simulink model "CIC2026_C1"  (R2025b)
settings: Solver=ode45  StartTime=0.0  StopTime=8000  FixedStep=0.1  RelTol=1e-3
StopFcn:
  | GuardaResultadoSimulacion;
model workspace (MATLAB code in the model file):
  | % 24 ºC
  | %%%%%%%%%%%%%%%%%%%%%%%%%%%%%%%%%%%%%%%%%%%%%%%%%%
  | Tev_Qev_24_75 = ...
  | [5.0,37.938;
  | 5.1,37.939 ;
  | 5.2,38.028 ;
  | 5.3,38.162 ;
  | 5.4,38.43  ;
  | 5.5,38.698 ;
  | 5.6,38.839 ;
  | 5.7,38.89  ;
  | 5.8,38.941 ;
  | 5.9,38.992 ;
  | 6,39.043   ;
  | 6.1,38.997 ;
  | 6.2,38.942 ;
  | 6.3,38.887 ;
  | 6.4,38.832 ;
  | 6.5,39.018 ;
  | 6.6,39.375 ;
  | 6.7,39.65  ;
  | 6.8,39.679 ;
  | 6.9,39.707 ;
  | 7,39.736   ;
  | 7.1,39.745 ;
  | 7.2,39.643 ;
  | 7.3,39.643 ;
  | 7.4,39.643 ;
  | 7.5,39.643 ;
  | 7.6,39.643 ;
  | 7.7,39.643 ;
  | 7.8,39.643 ;
  | 7.9,39.643 ;
  | 8,39.643   ;
  | 8.1,39.643 ;
  | 8.2,39.643 ;
  | 8.3,39.643 ;
  | 8.4,39.643 ;
  | 8.5,39.643 ;
  | 8.6,39.643 ;
  | 8.7,39.643 ;
  | 8.8,39.643 ;
  | 8.9,39.643 ;
  | 9,39.643   ;
  | 9.1,39.643 ;
  | 9.2,39.643 ;
  | 9.3,39.643 ;
  | 9.4,39.643 ;
  | 9.5,39.643 ;
  | 9.6,39.643 ;
  | 9.7,39.643 ;
  | 9.8,39.643 ;
  | 9.9,39.643 ;
  | 10,39.642  ;
  | 10.1,39.636;
  | 10.2,39.63 ;
  | 10.3,39.624;
  | 10.4,39.618;
  | 10.5,39.612;
  | 10.6,39.606;
  | 10.7,39.601;
  | 10.8,39.595;
  | 10.9,39.589;
  | 11,39.583  ;
  | 11.1,39.577;
  | 11.2,39.571;
  | 11.3,39.565;
  | 11.4,39.559;
  | 11.5,39.553;
  | 11.6,39.547;
  | 11.7,39.541;
  | 11.8,39.535;
  | 11.9,39.529;
  | 12.0,39.529];
  | 
  | Tev_Qev_24_80 = ...
  | [
  | 5.0,40.849   ;
  | 5.1,41.042   ;
  | 5.2,41.236   ;
  | 5.3,41.429   ;
  | 5.4,41.786   ;
  | 5.5,42.143   ;
  | 5.6,42.391   ;
  | 5.7,42.585   ;
  | 5.8,42.778   ;
  | 5.9,42.972   ;
  | 6,43.166     ;
  | 6.1,43.363   ;
  | 6.2,43.562   ;
  | 6.3,43.761   ;
  | 6.4,43.96    ;
  | 6.5,44.158   ;
  | 6.6,44.357   ;
  | 6.7,44.556   ;
  | 6.8,44.755   ;
  | 6.9,44.953   ;
  | 7,45.159     ;
  | 7.1,45.397   ;
  | 7.2,45.6     ;
  | 7.3,45.628   ;
  | 7.4,45.656   ;
  | 7.5,45.684   ;
  | 7.6,45.712   ;
  | 7.7,45.119   ;
  | 7.8,45.119   ;
  | 7.9,45.119   ;
  | 8,45.119     ;
  | 8.1,45.109   ;
  | 8.2,45.097   ;
  | 8.3,45.085   ;
  | 8.4,45.073   ;
  | 8.5,45.061   ;
  | 8.6,45.049   ;
  | 8.7,45.037   ;
  | 8.8,45.025   ;
  | 8.9,45.013   ;
  | 9,45.001     ;
  | 9.1,45.011   ;
  | 9.2,45.023   ;
  | 9.3,45.035   ;
  | 9.4,45.047   ;
  | 9.5,45.059   ;
  | 9.6,45.07    ;
  | 9.7,45.082   ;
  | 9.8,45.094   ;
  | 9.9,45.106   ;
  | 10,45.118    ;
  | 10.1,45.108  ;
  | 10.2,45.096  ;
  | 10.3,45.084  ;
  | 10.4,45.072  ;
  | 10.5,45.06   ;
  | 10.6,45.048  ;
  | 10.7,45.036  ;
  | 10.8,45.024  ;
  | 10.9,45.012  ;
  | 11,45        ;
  | 11.1,45.012  ;
  | 11.2,45.024  ;
  | 11.3,45.036  ;
  | 11.4,45.048  ;
  | 11.5,45.061  ;
  | 11.6,45.073  ;
  | 11.7,45.085  ;
  | 11.8,45.097  ;
  | 11.9,45.109  ;
  | 12.0,45.109
  | ];
  | 
  | Tev_Qev_24_85 = ...
  | [
  | 5.0,41.595   ;
  | 5.1,42.167   ;
  | 5.2,42.659   ;
  | 5.3,43.135   ;
  | 5.4,43.611   ;
  | 5.5,44.087   ;
  | 5.6,44.544   ;
  | 5.7,44.996   ;
  | 5.8,45.448   ;
  | 5.9,45.901   ;
  | 6,46.353     ;
  | 6.1,46.776   ;
  | 6.2,47.192   ;
  | 6.3,47.609   ;
  | 6.4,48.026   ;
  | 6.5,48.442   ;
  | 6.6,48.859   ;
  | 6.7,49.276   ;
  | 6.8,49.692   ;
  | 6.9,50       ;
  | 7,50.299     ;
  | 7.1,50.667   ;
  | 7.2,51.034   ;
  | 7.3,51.345   ;
  | 7.4,51.534   ;
  | 7.5,51.786   ;
  | 7.6,51.786   ;
  | 7.7,51.786   ;
  | 7.8,51.786   ;
  | 7.9,51.786   ;
  | 8,51.786     ;
  | 8.1,51.776   ;
  | 8.2,51.764   ;
  | 8.3,51.752   ;
  | 8.4,51.74    ;
  | 8.5,51.728   ;
  | 8.6,51.716   ;
  | 8.7,51.704   ;
  | 8.8,51.692   ;
  | 8.9,51.68    ;
  | 9,51.668     ;
  | 9.1,51.688   ;
  | 9.2,51.711   ;
  | 9.3,51.734   ;
  | 9.4,51.757   ;
  | 9.5,51.78    ;
  | 9.6,51.905   ;
  | 9.7,52.063   ;
  | 9.8,52.222   ;
  | 9.9,52.254   ;
  | 10,52.244    ;
  | 10.1,52.234  ;
  | 10.2,52.223  ;
  | 10.3,52.213  ;
  | 10.4,52.203  ;
  | 10.5,52.193  ;
  | 10.6,52.182  ;
  | 10.7,52.172  ;
  | 10.8,52.162  ;
  | 10.9,52.151  ;
  | 11,52.147    ;
  | 11.1,52.171  ;
  | 11.2,52.195  ;
  | 11.3,52.219  ;
  | 11.4,52.243  ;
  | 11.5,52.267  ;
  | 11.6,52.291  ;
  | 11.7,52.315  ;
  | 11.8,52.339  ;
  | 11.9,52.363  ;
  | 12.0,52.363
  | ];
  | 
  | Tev_Qev_24_88 = ...
  | [
  | 5,44.09      ;
  | 5.1,44.594   ;
  | 5.2,44.992   ;
  | 5.3,45.337   ;
  | 5.4,45.774   ;
  | 5.5,46.488   ;
  | 5.6,47.168   ;
  | 5.7,47.47    ;
  | 5.8,47.772   ;
  | 5.9,48.075   ;
  | 6,48.377     ;
  | 6.1,48.759   ;
  | 6.2,49.167   ;
  | 6.3,49.325   ;
  | 6.4,49.484   ;
  | 6.5,49.952   ;
  | 6.6,50.524   ;
  | 6.7,50.994   ;
  | 6.8,51.162   ;
  | 6.9,51.331   ;
  | 7,51.634     ;
  | 7.1,52.126   ;
  | 7.2,52.619   ;
  | 7.3,53.016   ;
  | 7.4,53.506   ;
  | 7.5,54.091   ;
  | 7.6,54.286   ;
  | 7.7,54.568   ;
  | 7.8,54.991   ;
  | 7.9,55.238   ;
  | 8,55.238     ;
  | 8.1,55.238   ;
  | 8.2,55.506   ;
  | 8.3,55.595   ;
  | 8.4,55.595   ;
  | 8.5,55.595   ;
  | 8.6,55.595   ;
  | 8.7,55.595   ;
  | 8.8,55.595   ;
  | 8.9,55.595   ;
  | 9,55.595     ;
  | 9.1,55.595   ;
  | 9.2,55.595   ;
  | 9.3,55.595   ;
  | 9.4,55.595   ;
  | 9.5,55.608   ;
  | 9.6,55.767   ;
  | 9.7,55.926   ;
  | 9.8,56.071   ;
  | 9.9,56.071   ;
  | 10,56.071    ;
  | 10.1,56.071  ;
  | 10.2,56.071  ;
  | 10.3,56.071  ;
  | 10.4,56.071  ;
  | 10.5,56.071  ;
  | 10.6,56.071  ;
  | 10.7,56.071  ;
  | 10.8,56.071  ;
  | 10.9,56.071  ;
  | 11,56.071    ;
  | 11.1,56.071  ;
  | 11.2,56.071  ;
  | 11.3,56.071  ;
  | 11.4,56.071  ;
  | 11.5,56.071  ;
  | 11.6,56.071  ;
  | 11.7,56.071  ;
  | 11.8,56.071  ;
  | 11.9,56.071  ;
  | 12.0,56.071
  | ];
  | 
  | Tev_Qev_24_95 = ...
  | [
  | 5,46.228     ;
  | 5.1,46.674   ;
  | 5.2,47.121   ;
  | 5.3,47.567   ;
  | 5.4,48.019   ;
  | 5.5,48.529   ;
  | 5.6,49.039   ;
  | 5.7,49.549   ;
  | 5.8,50.081   ;
  | 5.9,50.627   ;
  | 6,51.173     ;
  | 6.1,51.778   ;
  | 6.2,52.403   ;
  | 6.3,53.028   ;
  | 6.4,53.653   ;
  | 6.5,54.039   ;
  | 6.6,54.345   ;
  | 6.7,54.821   ;
  | 6.8,55.536   ;
  | 6.9,56.221   ;
  | 7,56.584     ;
  | 7.1,56.948   ;
  | 7.2,57.312   ;
  | 7.3,57.675   ;
  | 7.4,58       ;
  | 7.5,58.286   ;
  | 7.6,58.552   ;
  | 7.7,58.746   ;
  | 7.8,58.832   ;
  | 7.9,58.865   ;
  | 8,58.898     ;
  | 8.1,58.96    ;
  | 8.2,59.332   ;
  | 8.3,59.637   ;
  | 8.4,59.599   ;
  | 8.5,59.561   ;
  | 8.6,59.524   ;
  | 8.7,59.646   ;
  | 8.8,59.768   ;
  | 8.9,59.89    ;
  | 9,60.012     ;
  | 9.1,60.134   ;
  | 9.2,60.256   ;
  | 9.3,60.363   ;
  | 9.4,60.395   ;
  | 9.5,60.427   ;
  | 9.6,60.46    ;
  | 9.7,60.563   ;
  | 9.8,60.738   ;
  | 9.9,60.912   ;
  | 10,61.068    ;
  | 10.1,61.028  ;
  | 10.2,60.989  ;
  | 10.3,60.949  ;
  | 10.4,60.909  ;
  | 10.5,60.87   ;
  | 10.6,60.833  ;
  | 10.7,60.833  ;
  | 10.8,60.833  ;
  | 10.9,60.833  ;
  | 11,60.832    ;
  | 11.1,60.82   ;
  | 11.2,60.808  ;
  | 11.3,60.796  ;
  | 11.4,60.784  ;
  | 11.5,60.772  ;
  | 11.6,60.76   ;
  | 11.7,60.748  ;
  | 11.8,60.735  ;
  | 11.9,60.723  ;
  | 12.0,60.723
  | ];
  | 
  | Tev_COP_24_75 = ...
  | [
  | 5,0.704      ;
  | 5.1,0.708    ;
  | 5.2,0.712    ;
  | 5.3,0.716    ;
  | 5.4,0.72     ;
  | 5.5,0.724    ;
  | 5.6,0.728    ;
  | 5.7,0.732    ;
  | 5.8,0.736    ;
  | 5.9,0.74     ;
  | 6,0.743      ;
  | 6.1,0.747    ;
  | 6.2,0.752    ;
  | 6.3,0.758    ;
  | 6.4,0.765    ;
  | 6.5,0.77     ;
  | 6.6,0.774    ;
  | 6.7,0.777    ;
  | 6.8,0.779    ;
  | 6.9,0.781    ;
  | 7,0.788      ;
  | 7.1,0.794    ;
  | 7.2,0.796    ;
  | 7.3,0.796    ;
  | 7.4,0.796    ;
  | 7.5,0.796    ;
  | 7.6,0.796    ;
  | 7.7,0.796    ;
  | 7.8,0.796    ;
  | 7.9,0.796    ;
  | 8,0.796      ;
  | 8.1,0.796    ;
  | 8.2,0.796    ;
  | 8.3,0.796    ;
  | 8.4,0.796    ;
  | 8.5,0.797    ;
  | 8.6,0.797    ;
  | 8.7,0.797    ;
  | 8.8,0.797    ;
  | 8.9,0.797    ;
  | 9,0.797      ;
  | 9.1,0.797    ;
  | 9.2,0.797    ;
  | 9.3,0.797    ;
  | 9.4,0.797    ;
  | 9.5,0.797    ;
  | 9.6,0.797    ;
  | 9.7,0.797    ;
  | 9.8,0.797    ;
  | 9.9,0.797    ;
  | 10,0.797     ;
  | 10.1,0.797   ;
  | 10.2,0.798   ;
  | 10.3,0.798   ;
  | 10.4,0.798   ;
  | 10.5,0.798   ;
  | 10.6,0.798   ;
  | 10.7,0.798   ;
  | 10.8,0.798   ;
  | 10.9,0.798   ;
  | 11,0.798     ;
  | 11.1,0.798   ;
  | 11.2,0.798   ;
  | 11.3,0.798   ;
  | 11.4,0.798   ;
  | 11.5,0.798   ;
  | 11.6,0.798   ;
  | 11.7,0.798   ;
  | 11.8,0.798   ;
  | 11.9,0.799   ;
  | 12.0,0.799
  | ];
  | 
  | Tev_COP_24_80 = ...
  | [
  | 5,0.671      ;
  | 5.1,0.677    ;
  | 5.2,0.682    ;
  | 5.3,0.688    ;
  | 5.4,0.693    ;
  | 5.5,0.699    ;
  | 5.6,0.704    ;
  | 5.7,0.709    ;
  | 5.8,0.714    ;
  | 5.9,0.719    ;
  | 6,0.724      ;
  | 6.1,0.728    ;
  | 6.2,0.733    ;
  | 6.3,0.739    ;
  | 6.4,0.743    ;
  | 6.5,0.748    ;
  | 6.6,0.752    ;
  | 6.7,0.758    ;
  | 6.8,0.763    ;
  | 6.9,0.767    ;
  | 7,0.77       ;
  | 7.1,0.773    ;
  | 7.2,0.774    ;
  | 7.3,0.775    ;
  | 7.4,0.775    ;
  | 7.5,0.775    ;
  | 7.6,0.775    ;
  | 7.7,0.776    ;
  | 7.8,0.769    ;
  | 7.9,0.769    ;
  | 8,0.77       ;
  | 8.1,0.77     ;
  | 8.2,0.77     ;
  | 8.3,0.77     ;
  | 8.4,0.769    ;
  | 8.5,0.769    ;
  | 8.6,0.769    ;
  | 8.7,0.769    ;
  | 8.8,0.769    ;
  | 8.9,0.769    ;
  | 9,0.769      ;
  | 9.1,0.769    ;
  | 9.2,0.769    ;
  | 9.3,0.769    ;
  | 9.4,0.769    ;
  | 9.5,0.769    ;
  | 9.6,0.769    ;
  | 9.7,0.77     ;
  | 9.8,0.77     ;
  | 9.9,0.77     ;
  | 10,0.77      ;
  | 10.1,0.77    ;
  | 10.2,0.77    ;
  | 10.3,0.77    ;
  | 10.4,0.77    ;
  | 10.5,0.77    ;
  | 10.6,0.77    ;
  | 10.7,0.77    ;
  | 10.8,0.77    ;
  | 10.9,0.77    ;
  | 11,0.77      ;
  | 11.1,0.77    ;
  | 11.2,0.77    ;
  | 11.3,0.77    ;
  | 11.4,0.771   ;
  | 11.5,0.771   ;
  | 11.6,0.771   ;
  | 11.7,0.771   ;
  | 11.8,0.771   ;
  | 11.9,0.771   ;
  | 12.0,0.771
  | ];
  | 
  | Tev_COP_24_85 = ...
  | [
  | 5,0.616      ;
  | 5.1,0.622    ;
  | 5.2,0.629    ;
  | 5.3,0.635    ;
  | 5.4,0.641    ;
  | 5.5,0.648    ;
  | 5.6,0.654    ;
  | 5.7,0.66     ;
  | 5.8,0.666    ;
  | 5.9,0.671    ;
  | 6,0.675      ;
  | 6.1,0.68     ;
  | 6.2,0.686    ;
  | 6.3,0.691    ;
  | 6.4,0.697    ;
  | 6.5,0.702    ;
  | 6.6,0.708    ;
  | 6.7,0.713    ;
  | 6.8,0.719    ;
  | 6.9,0.724    ;
  | 7,0.73       ;
  | 7.1,0.734    ;
  | 7.2,0.738    ;
  | 7.3,0.741    ;
  | 7.4,0.742    ;
  | 7.5,0.742    ;
  | 7.6,0.742    ;
  | 7.7,0.742    ;
  | 7.8,0.742    ;
  | 7.9,0.743    ;
  | 8,0.743      ;
  | 8.1,0.743    ;
  | 8.2,0.743    ;
  | 8.3,0.742    ;
  | 8.4,0.742    ;
  | 8.5,0.742    ;
  | 8.6,0.742    ;
  | 8.7,0.742    ;
  | 8.8,0.742    ;
  | 8.9,0.742    ;
  | 9,0.743      ;
  | 9.1,0.745    ;
  | 9.2,0.746    ;
  | 9.3,0.746    ;
  | 9.4,0.747    ;
  | 9.5,0.747    ;
  | 9.6,0.747    ;
  | 9.7,0.748    ;
  | 9.8,0.748    ;
  | 9.9,0.748    ;
  | 10,0.749     ;
  | 10.1,0.748   ;
  | 10.2,0.748   ;
  | 10.3,0.748   ;
  | 10.4,0.748   ;
  | 10.5,0.748   ;
  | 10.6,0.748   ;
  | 10.7,0.748   ;
  | 10.8,0.747   ;
  | 10.9,0.747   ;
  | 11,0.747     ;
  | 11.1,0.747   ;
  | 11.2,0.747   ;
  | 11.3,0.748   ;
  | 11.4,0.748   ;
  | 11.5,0.748   ;
  | 11.6,0.748   ;
  | 11.7,0.748   ;
  | 11.8,0.748   ;
  | 11.9,0.748   ;
  | 12.0,0.748
  | ];
  | 
  | Tev_COP_24_88 = ...
  | [
  | 5,0.601      ;
  | 5.1,0.605    ;
  | 5.2,0.609    ;
  | 5.3,0.613    ;
  | 5.4,0.617    ;
  | 5.5,0.62     ;
  | 5.6,0.624    ;
  | 5.7,0.629    ;
  | 5.8,0.635    ;
  | 5.9,0.64     ;
  | 6,0.646      ;
  | 6.1,0.651    ;
  | 6.2,0.656    ;
  | 6.3,0.66     ;
  | 6.4,0.665    ;
  | 6.5,0.671    ;
  | 6.6,0.678    ;
  | 6.7,0.685    ;
  | 6.8,0.69     ;
  | 6.9,0.695    ;
  | 7,0.7        ;
  | 7.1,0.701    ;
  | 7.2,0.701    ;
  | 7.3,0.704    ;
  | 7.4,0.709    ;
  | 7.5,0.705    ;
  | 7.6,0.703    ;
  | 7.7,0.703    ;
  | 7.8,0.702    ;
  | 7.9,0.702    ;
  | 8,0.702      ;
  | 8.1,0.702    ;
  | 8.2,0.701    ;
  | 8.3,0.701    ;
  | 8.4,0.701    ;
  | 8.5,0.701    ;
  | 8.6,0.701    ;
  | 8.7,0.7      ;
  | 8.8,0.7      ;
  | 8.9,0.702    ;
  | 9,0.705      ;
  | 9.1,0.708    ;
  | 9.2,0.708    ;
  | 9.3,0.708    ;
  | 9.4,0.708    ;
  | 9.5,0.708    ;
  | 9.6,0.708    ;
  | 9.7,0.708    ;
  | 9.8,0.707    ;
  | 9.9,0.707    ;
  | 10,0.707     ;
  | 10.1,0.707   ;
  | 10.2,0.707   ;
  | 10.3,0.707   ;
  | 10.4,0.707   ;
  | 10.5,0.707   ;
  | 10.6,0.707   ;
  | 10.7,0.707   ;
  | 10.8,0.707   ;
  | 10.9,0.707   ;
  | 11,0.707     ;
  | 11.1,0.707   ;
  | 11.2,0.707   ;
  | 11.3,0.708   ;
  | 11.4,0.708   ;
  | 11.5,0.708   ;
  | 11.6,0.708   ;
  | 11.7,0.708   ;
  | 11.8,0.708   ;
  | 11.9,0.708   ;
  | 12.0,0.708
  | ];
  | 
  | Tev_COP_24_95 = ...
  | [
  | 5,0.54        ;
  | 5.1,0.547     ;
  | 5.2,0.555     ;
  | 5.3,0.562     ;
  | 5.4,0.563     ;
  | 5.5,0.565     ;
  | 5.6,0.57      ;
  | 5.7,0.577     ;
  | 5.8,0.584     ;
  | 5.9,0.591     ;
  | 6,0.598       ;
  | 6.1,0.605     ;
  | 6.2,0.609     ;
  | 6.3,0.613     ;
  | 6.4,0.617     ;
  | 6.5,0.621     ;
  | 6.6,0.624     ;
  | 6.7,0.629     ;
  | 6.8,0.638     ;
  | 6.9,0.646     ;
  | 7,0.651       ;
  | 7.1,0.657     ;
  | 7.2,0.662     ;
  | 7.3,0.663     ;
  | 7.4,0.667     ;
  | 7.5,0.672     ;
  | 7.6,0.679     ;
  | 7.7,0.68      ;
  | 7.8,0.68      ;
  | 7.9,0.681     ;
  | 8,0.685       ;
  | 8.1,0.686     ;
  | 8.2,0.686     ;
  | 8.3,0.686     ;
  | 8.4,0.687     ;
  | 8.5,0.687     ;
  | 8.6,0.687     ;
  | 8.7,0.689     ;
  | 8.8,0.691     ;
  | 8.9,0.693     ;
  | 9,0.692       ;
  | 9.1,0.692     ;
  | 9.2,0.691     ;
  | 9.3,0.691     ;
  | 9.4,0.69      ;
  | 9.5,0.689     ;
  | 9.6,0.689     ;
  | 9.7,0.69      ;
  | 9.8,0.692     ;
  | 9.9,0.694     ;
  | 10,0.696      ;
  | 10.1,0.696    ;
  | 10.2,0.695    ;
  | 10.3,0.695    ;
  | 10.4,0.695    ;
  | 10.5,0.695    ;
  | 10.6,0.695    ;
  | 10.7,0.695    ;
  | 10.8,0.695    ;
  | 10.9,0.694    ;
  | 11,0.694      ;
  | 11.1,0.694    ;
  | 11.2,0.694    ;
  | 11.3,0.694    ;
  | 11.4,0.694    ;
  | 11.5,0.694    ;
  | 11.6,0.694    ;
  | 11.7,0.694    ;
  | 11.8,0.694    ;
  | 11.9,0.694    ;
  | 12.0,0.694
  | ];
  | 
  | 
  | % 29 ºC
  | %%%%%%%%%%%%%%%%%%%%%%%%%%%%%%%%%%%%%%%%%%%%%%%%%%
  | Tev_Qev_29_75 = ...
  | [
  | 5,20.985      ;
  | 5.1,21.03     ;
  | 5.2,21.05     ;
  | 5.3,21.069    ;
  | 5.4,21.089    ;
  | 5.5,21.109    ;
  | 5.6,21.128    ;
  | 5.7,21.186    ;
  | 5.8,21.247    ;
  | 5.9,21.308    ;
  | 6,21.366      ;
  | 6.1,21.366    ;
  | 6.2,21.366    ;
  | 6.3,21.366    ;
  | 6.4,21.366    ;
  | 6.5,21.366    ;
  | 6.6,21.366    ;
  | 6.7,21.425    ;
  | 6.8,21.734    ;
  | 6.9,22.044    ;
  | 7,22.074      ;
  | 7.1,22.074    ;
  | 7.2,22.063    ;
  | 7.3,22.049    ;
  | 7.4,22.036    ;
  | 7.5,22.023    ;
  | 7.6,22.009    ;
  | 7.7,21.996    ;
  | 7.8,21.983    ;
  | 7.9,21.969    ;
  | 8,21.956      ;
  | 8.1,21.92     ;
  | 8.2,21.885    ;
  | 8.3,21.85     ;
  | 8.4,21.814    ;
  | 8.5,21.779    ;
  | 8.6,21.744    ;
  | 8.7,21.708    ;
  | 8.8,21.673    ;
  | 8.9,21.638    ;
  | 9,21.602      ;
  | 9.1,21.626    ;
  | 9.2,21.65     ;
  | 9.3,21.674    ;
  | 9.4,21.698    ;
  | 9.5,21.722    ;
  | 9.6,21.747    ;
  | 9.7,21.771    ;
  | 9.8,21.795    ;
  | 9.9,21.819    ;
  | 10,21.84      ;
  | 10.1,21.852   ;
  | 10.2,21.864   ;
  | 10.3,21.876   ;
  | 10.4,21.887   ;
  | 10.5,21.899   ;
  | 10.6,21.911   ;
  | 10.7,21.922   ;
  | 10.8,21.934   ;
  | 10.9,21.946   ;
  | 11,21.956     ;
  | 11.1,21.956   ;
  | 11.2,21.956   ;
  | 11.3,21.956   ;
  | 11.4,21.956   ;
  | 11.5,21.956   ;
  | 11.6,21.956   ;
  | 11.7,21.956   ;
  | 11.8,21.956   ;
  | 11.9,21.956   ;
  | 12,21.946
  | ];
  | 
  | Tev_Qev_29_80 = ...
  | [
  | 5,26.088      ;
  | 5.1,26.243    ;
  | 5.2,26.399    ;
  | 5.3,26.554    ;
  | 5.4,26.71     ;
  | 5.5,26.865    ;
  | 5.6,27.021    ;
  | 5.7,27.177    ;
  | 5.8,27.332    ;
  | 5.9,27.488    ;
  | 6,27.652      ;
  | 6.1,27.872    ;
  | 6.2,28.093    ;
  | 6.3,28.313    ;
  | 6.4,28.533    ;
  | 6.5,28.754    ;
  | 6.6,28.974    ;
  | 6.7,29.194    ;
  | 6.8,29.415    ;
  | 6.9,29.635    ;
  | 7,29.855      ;
  | 7.1,29.865    ;
  | 7.2,29.865    ;
  | 7.3,29.865    ;
  | 7.4,29.865    ;
  | 7.5,29.865    ;
  | 7.6,29.865    ;
  | 7.7,29.865    ;
  | 7.8,29.865    ;
  | 7.9,29.865    ;
  | 8,29.865      ;
  | 8.1,29.865    ;
  | 8.2,29.865    ;
  | 8.3,29.865    ;
  | 8.4,29.865    ;
  | 8.5,29.865    ;
  | 8.6,29.865    ;
  | 8.7,29.865    ;
  | 8.8,29.865    ;
  | 8.9,29.865    ;
  | 9,29.865      ;
  | 9.1,29.865    ;
  | 9.2,29.865    ;
  | 9.3,29.865    ;
  | 9.4,29.865    ;
  | 9.5,29.865    ;
  | 9.6,29.865    ;
  | 9.7,29.865    ;
  | 9.8,29.865    ;
  | 9.9,29.865    ;
  | 10,29.864     ;
  | 10.1,29.852   ;
  | 10.2,29.84    ;
  | 10.3,29.828   ;
  | 10.4,29.817   ;
  | 10.5,29.805   ;
  | 10.6,29.793   ;
  | 10.7,29.781   ;
  | 10.8,29.769   ;
  | 10.9,29.758   ;
  | 11,29.746     ;
  | 11.1,29.734   ;
  | 11.2,29.722   ;
  | 11.3,29.711   ;
  | 11.4,29.699   ;
  | 11.5,29.687   ;
  | 11.6,29.675   ;
  | 11.7,29.663   ;
  | 11.8,29.652   ;
  | 11.9,29.64    ;
  | 12,29.629
  | ];
  | 
  | Tev_Qev_29_85 = ...
  | [
  | 5,27.071      ;
  | 5.1,27.57     ;
  | 5.2,28.043    ;
  | 5.3,28.504    ;
  | 5.4,29.053    ;
  | 5.5,29.661    ;
  | 5.6,30.258    ;
  | 5.7,30.737    ;
  | 5.8,31.215    ;
  | 5.9,31.694    ;
  | 6,32.161      ;
  | 6.1,32.551    ;
  | 6.2,32.941    ;
  | 6.3,33.331    ;
  | 6.4,33.722    ;
  | 6.5,34.112    ;
  | 6.6,34.577    ;
  | 6.7,34.972    ;
  | 6.8,35.331    ;
  | 6.9,35.707    ;
  | 7,36.089      ;
  | 7.1,36.471    ;
  | 7.2,36.817    ;
  | 7.3,36.603    ;
  | 7.4,37.299    ;
  | 7.5,37.279    ;
  | 7.6,37.26     ;
  | 7.7,37.241    ;
  | 7.8,37.222    ;
  | 7.9,37.203    ;
  | 8,37.184      ;
  | 8.1,37.17     ;
  | 8.2,37.157    ;
  | 8.3,37.144    ;
  | 8.4,37.13     ;
  | 8.5,37.117    ;
  | 8.6,37.104    ;
  | 8.7,37.09     ;
  | 8.8,37.077    ;
  | 8.9,37.097    ;
  | 9,37.278      ;
  | 9.1,37.46     ;
  | 9.2,37.528    ;
  | 9.3,37.511    ;
  | 9.4,37.494    ;
  | 9.5,37.477    ;
  | 9.6,37.46     ;
  | 9.7,37.443    ;
  | 9.8,37.426    ;
  | 9.9,37.589    ;
  | 10,37.861     ;
  | 10.1,37.903   ;
  | 10.2,37.914   ;
  | 10.3,37.926   ;
  | 10.4,37.938   ;
  | 10.5,37.95    ;
  | 10.6,37.962   ;
  | 10.7,37.974   ;
  | 10.8,37.986   ;
  | 10.9,37.998   ;
  | 11,38.009     ;
  | 11.1,38.033   ;
  | 11.2,38.057   ;
  | 11.3,38.081   ;
  | 11.4,38.104   ;
  | 11.5,38.128   ;
  | 11.6,38.152   ;
  | 11.7,38.176   ;
  | 11.8,38.2     ;
  | 11.9,38.224   ;
  | 12,38.236
  | ];
  | 
  | Tev_Qev_29_88 = ...
  | [
  | 5,34.256       ;
  | 5.1,34.835     ;
  | 5.2,35.201     ;
  | 5.3,35.519     ;
  | 5.4,35.837     ;
  | 5.5,36.149     ;
  | 5.6,36.402     ;
  | 5.7,36.655     ;
  | 5.8,36.908     ;
  | 5.9,37.161     ;
  | 6,37.414       ;
  | 6.1,37.745     ;
  | 6.2,38.077     ;
  | 6.3,38.41      ;
  | 6.4,38.742     ;
  | 6.5,39.074     ;
  | 6.6,39.407     ;
  | 6.7,39.739     ;
  | 6.8,40.217     ;
  | 6.9,40.716     ;
  | 7,41.082       ;
  | 7.1,41.402     ;
  | 7.2,41.723     ;
  | 7.3,41.959     ;
  | 7.4,42.505     ;
  | 7.5,42.808     ;
  | 7.6,43.161     ;
  | 7.7,43.25      ;
  | 7.8,43.453     ;
  | 7.9,43.917     ;
  | 8,44.255       ;
  | 8.1,44.21      ;
  | 8.2,44.165     ;
  | 8.3,44.209     ;
  | 8.4,44.302     ;
  | 8.5,44.39      ;
  | 8.6,44.437     ;
  | 8.7,44.484     ;
  | 8.8,44.53      ;
  | 8.9,44.577     ;
  | 9,44.62        ;
  | 9.1,44.605     ;
  | 9.2,44.591     ;
  | 9.3,44.576     ;
  | 9.4,44.562     ;
  | 9.5,44.548     ;
  | 9.6,44.533     ;
  | 9.7,44.519     ;
  | 9.8,44.505     ;
  | 9.9,44.645     ;
  | 10,44.812      ;
  | 10.1,44.875    ;
  | 10.2,44.899    ;
  | 10.3,44.924    ;
  | 10.4,44.948    ;
  | 10.5,44.973    ;
  | 10.6,44.997    ;
  | 10.7,45.022    ;
  | 10.8,45.046    ;
  | 10.9,45.071    ;
  | 11,45.092      ;
  | 11.1,45.08     ;
  | 11.2,45.068    ;
  | 11.3,45.056    ;
  | 11.4,45.044    ;
  | 11.5,45.032    ;
  | 11.6,45.02     ;
  | 11.7,45.008    ;
  | 11.8,44.996    ;
  | 11.9,44.984    ;
  | 12,45
  | ];
  | 
  | Tev_Qev_29_95 = ...
  | [
  | 5,39.362       ;
  | 5.1,40.037     ;
  | 5.2,40.713     ;
  | 5.3,41.131     ;
  | 5.4,41.399     ;
  | 5.5,41.668     ;
  | 5.6,42.056     ;
  | 5.7,42.541     ;
  | 5.8,43.025     ;
  | 5.9,43.51      ;
  | 6,43.994       ;
  | 6.1,44.479     ;
  | 6.2,44.796     ;
  | 6.3,45.104     ;
  | 6.4,45.411     ;
  | 6.5,45.719     ;
  | 6.6,46.027     ;
  | 6.7,46.424     ;
  | 6.8,46.883     ;
  | 6.9,47.342     ;
  | 7,47.8         ;
  | 7.1,48.259     ;
  | 7.2,48.718     ;
  | 7.3,49.177     ;
  | 7.4,49.266     ;
  | 7.5,49.146     ;
  | 7.6,49.742     ;
  | 7.7,49.897     ;
  | 7.8,49.853     ;
  | 7.9,49.809     ;
  | 8,49.765       ;
  | 8.1,49.721     ;
  | 8.2,49.946     ;
  | 8.3,50.314     ;
  | 8.4,50.382     ;
  | 8.5,50.593     ;
  | 8.6,50.746     ;
  | 8.7,50.715     ;
  | 8.8,50.684     ;
  | 8.9,50.653     ;
  | 9,50.726       ;
  | 9.1,50.864     ;
  | 9.2,51.003     ;
  | 9.3,51.141     ;
  | 9.4,51.279     ;
  | 9.5,51.417     ;
  | 9.6,51.555     ;
  | 9.7,51.693     ;
  | 9.8,51.831     ;
  | 9.9,51.969     ;
  | 10,52.053      ;
  | 10.1,52.04     ;
  | 10.2,52.027    ;
  | 10.3,52.014    ;
  | 10.4,52.001    ;
  | 10.5,51.988    ;
  | 10.6,51.975    ;
  | 10.7,51.962    ;
  | 10.8,51.949    ;
  | 10.9,52.065    ;
  | 11,52.505      ;
  | 11.1,52.594    ;
  | 11.2,52.585    ;
  | 11.3,52.286    ;
  | 11.4,52.164    ;
  | 11.5,52.146    ;
  | 11.6,52.128    ;
  | 11.7,52.11     ;
  | 11.8,52.092    ;
  | 11.9,52.074    ;
  | 12,52.057
  | ];
  | 
  | Tev_COP_29_75 = ...
  | [
  | 5,0.666        ;
  | 5.1,0.671      ;
  | 5.2,0.676      ;
  | 5.3,0.681      ;
  | 5.4,0.686      ;
  | 5.5,0.691      ;
  | 5.6,0.696      ;
  | 5.7,0.701      ;
  | 5.8,0.704      ;
  | 5.9,0.708      ;
  | 6,0.712        ;
  | 6.1,0.716      ;
  | 6.2,0.721      ;
  | 6.3,0.726      ;
  | 6.4,0.731      ;
  | 6.5,0.734      ;
  | 6.6,0.736      ;
  | 6.7,0.738      ;
  | 6.8,0.74       ;
  | 6.9,0.743      ;
  | 7,0.749        ;
  | 7.1,0.755      ;
  | 7.2,0.755      ;
  | 7.3,0.755      ;
  | 7.4,0.755      ;
  | 7.5,0.755      ;
  | 7.6,0.755      ;
  | 7.7,0.754      ;
  | 7.8,0.754      ;
  | 7.9,0.754      ;
  | 8,0.754        ;
  | 8.1,0.754      ;
  | 8.2,0.754      ;
  | 8.3,0.754      ;
  | 8.4,0.753      ;
  | 8.5,0.753      ;
  | 8.6,0.753      ;
  | 8.7,0.753      ;
  | 8.8,0.753      ;
  | 8.9,0.753      ;
  | 9,0.753        ;
  | 9.1,0.753      ;
  | 9.2,0.753      ;
  | 9.3,0.753      ;
  | 9.4,0.753      ;
  | 9.5,0.753      ;
  | 9.6,0.753      ;
  | 9.7,0.753      ;
  | 9.8,0.753      ;
  | 9.9,0.753      ;
  | 10,0.753       ;
  | 10.1,0.753     ;
  | 10.2,0.753     ;
  | 10.3,0.753     ;
  | 10.4,0.754     ;
  | 10.5,0.754     ;
  | 10.6,0.754     ;
  | 10.7,0.755     ;
  | 10.8,0.755     ;
  | 10.9,0.755     ;
  | 11,0.755       ;
  | 11.1,0.755     ;
  | 11.2,0.755     ;
  | 11.3,0.754     ;
  | 11.4,0.754     ;
  | 11.5,0.754     ;
  | 11.6,0.754     ;
  | 11.7,0.753     ;
  | 11.8,0.753     ;
  | 11.9,0.753     ;
  | 12,0.753
  | ];
  | 
  | Tev_COP_29_80 = ...
  | [
  | 5,0.65         ;
  | 5.1,0.652      ;
  | 5.2,0.655      ;
  | 5.3,0.658      ;
  | 5.4,0.666      ;
  | 5.5,0.674      ;
  | 5.6,0.68       ;
  | 5.7,0.683      ;
  | 5.8,0.687      ;
  | 5.9,0.691      ;
  | 6,0.694        ;
  | 6.1,0.699      ;
  | 6.2,0.704      ;
  | 6.3,0.708      ;
  | 6.4,0.713      ;
  | 6.5,0.718      ;
  | 6.6,0.723      ;
  | 6.7,0.728      ;
  | 6.8,0.732      ;
  | 6.9,0.738      ;
  | 7,0.742        ;
  | 7.1,0.74       ;
  | 7.2,0.743      ;
  | 7.3,0.746      ;
  | 7.4,0.746      ;
  | 7.5,0.746      ;
  | 7.6,0.741      ;
  | 7.7,0.741      ;
  | 7.8,0.741      ;
  | 7.9,0.741      ;
  | 8,0.741        ;
  | 8.1,0.741      ;
  | 8.2,0.741      ;
  | 8.3,0.741      ;
  | 8.4,0.742      ;
  | 8.5,0.742      ;
  | 8.6,0.742      ;
  | 8.7,0.742      ;
  | 8.8,0.742      ;
  | 8.9,0.742      ;
  | 9,0.742        ;
  | 9.1,0.742      ;
  | 9.2,0.742      ;
  | 9.3,0.742      ;
  | 9.4,0.742      ;
  | 9.5,0.742      ;
  | 9.6,0.742      ;
  | 9.7,0.741      ;
  | 9.8,0.741      ;
  | 9.9,0.741      ;
  | 10,0.741       ;
  | 10.1,0.741     ;
  | 10.2,0.741     ;
  | 10.3,0.741     ;
  | 10.4,0.74      ;
  | 10.5,0.74      ;
  | 10.6,0.74      ;
  | 10.7,0.74      ;
  | 10.8,0.74      ;
  | 10.9,0.74      ;
  | 11,0.74        ;
  | 11.1,0.74      ;
  | 11.2,0.74      ;
  | 11.3,0.74      ;
  | 11.4,0.74      ;
  | 11.5,0.74      ;
  | 11.6,0.74      ;
  | 11.7,0.741     ;
  | 11.8,0.741     ;
  | 11.9,0.741     ;
  | 12,0.741
  | ];
  | 
  | Tev_COP_29_85 = ...
  | [
  | 5,0.627        ;
  | 5.1,0.632      ;
  | 5.2,0.638      ;
  | 5.3,0.644      ;
  | 5.4,0.648      ;
  | 5.5,0.652      ;
  | 5.6,0.656      ;
  | 5.7,0.66       ;
  | 5.8,0.665      ;
  | 5.9,0.67       ;
  | 6,0.675        ;
  | 6.1,0.679      ;
  | 6.2,0.684      ;
  | 6.3,0.688      ;
  | 6.4,0.693      ;
  | 6.5,0.696      ;
  | 6.6,0.699      ;
  | 6.7,0.704      ;
  | 6.8,0.709      ;
  | 6.9,0.714      ;
  | 7,0.718        ;
  | 7.1,0.721      ;
  | 7.2,0.724      ;
  | 7.3,0.727      ;
  | 7.4,0.727      ;
  | 7.5,0.727      ;
  | 7.6,0.727      ;
  | 7.7,0.727      ;
  | 7.8,0.728      ;
  | 7.9,0.728      ;
  | 8,0.728        ;
  | 8.1,0.728      ;
  | 8.2,0.727      ;
  | 8.3,0.727      ;
  | 8.4,0.731      ;
  | 8.5,0.733      ;
  | 8.6,0.733      ;
  | 8.7,0.734      ;
  | 8.8,0.734      ;
  | 8.9,0.735      ;
  | 9,0.735        ;
  | 9.1,0.735      ;
  | 9.2,0.735      ;
  | 9.3,0.735      ;
  | 9.4,0.735      ;
  | 9.5,0.735      ;
  | 9.6,0.734      ;
  | 9.7,0.734      ;
  | 9.8,0.734      ;
  | 9.9,0.734      ;
  | 10,0.734       ;
  | 10.1,0.734     ;
  | 10.2,0.735     ;
  | 10.3,0.735     ;
  | 10.4,0.736     ;
  | 10.5,0.736     ;
  | 10.6,0.737     ;
  | 10.7,0.737     ;
  | 10.8,0.737     ;
  | 10.9,0.738     ;
  | 11,0.738       ;
  | 11.1,0.738     ;
  | 11.2,0.738     ;
  | 11.3,0.739     ;
  | 11.4,0.739     ;
  | 11.5,0.739     ;
  | 11.6,0.739     ;
  | 11.7,0.739     ;
  | 11.8,0.739     ;
  | 11.9,0.739     ;
  | 12,0.739
  | ];
  | 
  | Tev_COP_29_88 = ...
  | [
  | 5,0.615        ;
  | 5.1,0.619      ;
  | 5.2,0.624      ;
  | 5.3,0.628      ;
  | 5.4,0.634      ;
  | 5.5,0.641      ;
  | 5.6,0.648      ;
  | 5.7,0.652      ;
  | 5.8,0.657      ;
  | 5.9,0.661      ;
  | 6,0.666        ;
  | 6.1,0.67       ;
  | 6.2,0.675      ;
  | 6.3,0.684      ;
  | 6.4,0.691      ;
  | 6.5,0.694      ;
  | 6.6,0.696      ;
  | 6.7,0.699      ;
  | 6.8,0.704      ;
  | 6.9,0.708      ;
  | 7,0.713        ;
  | 7.1,0.718      ;
  | 7.2,0.722      ;
  | 7.3,0.727      ;
  | 7.4,0.728      ;
  | 7.5,0.721      ;
  | 7.6,0.723      ;
  | 7.7,0.715      ;
  | 7.8,0.715      ;
  | 7.9,0.715      ;
  | 8,0.715        ;
  | 8.1,0.715      ;
  | 8.2,0.715      ;
  | 8.3,0.716      ;
  | 8.4,0.721      ;
  | 8.5,0.723      ;
  | 8.6,0.723      ;
  | 8.7,0.722      ;
  | 8.8,0.721      ;
  | 8.9,0.723      ;
  | 9,0.726        ;
  | 9.1,0.728      ;
  | 9.2,0.728      ;
  | 9.3,0.728      ;
  | 9.4,0.728      ;
  | 9.5,0.728      ;
  | 9.6,0.728      ;
  | 9.7,0.728      ;
  | 9.8,0.728      ;
  | 9.9,0.728      ;
  | 10,0.728       ;
  | 10.1,0.728     ;
  | 10.2,0.728     ;
  | 10.3,0.728     ;
  | 10.4,0.727     ;
  | 10.5,0.727     ;
  | 10.6,0.727     ;
  | 10.7,0.727     ;
  | 10.8,0.727     ;
  | 10.9,0.727     ;
  | 11,0.727       ;
  | 11.1,0.727     ;
  | 11.2,0.727     ;
  | 11.3,0.727     ;
  | 11.4,0.727     ;
  | 11.5,0.727     ;
  | 11.6,0.727     ;
  | 11.7,0.728     ;
  | 11.8,0.728     ;
  | 11.9,0.728     ;
  | 12,0.728
  | ];
  | 
  | Tev_COP_29_95 = ...
  | [
  | 5,0.567        ;
  | 5.1,0.574      ;
  | 5.2,0.58       ;
  | 5.3,0.587      ;
  | 5.4,0.594      ;
  | 5.5,0.6        ;
  | 5.6,0.606      ;
  | 5.7,0.612      ;
  | 5.8,0.618      ;
  | 5.9,0.624      ;
  | 6,0.63         ;
  | 6.1,0.636      ;
  | 6.2,0.643      ;
  | 6.3,0.649      ;
  | 6.4,0.656      ;
  | 6.5,0.662      ;
  | 6.6,0.668      ;
  | 6.7,0.675      ;
  | 6.8,0.683      ;
  | 6.9,0.69       ;
  | 7,0.691        ;
  | 7.1,0.693      ;
  | 7.2,0.695      ;
  | 7.3,0.703      ;
  | 7.4,0.707      ;
  | 7.5,0.711      ;
  | 7.6,0.711      ;
  | 7.7,0.711      ;
  | 7.8,0.712      ;
  | 7.9,0.712      ;
  | 8,0.712        ;
  | 8.1,0.712      ;
  | 8.2,0.712      ;
  | 8.3,0.712      ;
  | 8.4,0.712      ;
  | 8.5,0.712      ;
  | 8.6,0.711      ;
  | 8.7,0.711      ;
  | 8.8,0.711      ;
  | 8.9,0.711      ;
  | 9,0.711        ;
  | 9.1,0.711      ;
  | 9.2,0.711      ;
  | 9.3,0.711      ;
  | 9.4,0.711      ;
  | 9.5,0.712      ;
  | 9.6,0.712      ;
  | 9.7,0.712      ;
  | 9.8,0.712      ;
  | 9.9,0.712      ;
  | 10,0.712       ;
  | 10.1,0.712     ;
  | 10.2,0.712     ;
  | 10.3,0.712     ;
  | 10.4,0.712     ;
  | 10.5,0.712     ;
  | 10.6,0.712     ;
  | 10.7,0.712     ;
  | 10.8,0.712     ;
  | 10.9,0.712     ;
  | 11,0.712       ;
  | 11.1,0.712     ;
  | 11.2,0.712     ;
  | 11.3,0.712     ;
  | 11.4,0.712     ;
  | 11.5,0.712     ;
  | 11.6,0.711     ;
  | 11.7,0.711     ;
  | 11.8,0.711     ;
  | 11.9,0.711     ;
  | 12,0.711
  | ];
  | 
  | 
  | % 31 ºC
  | %%%%%%%%%%%%%%%%%%%%%%%%%%%%%%%%%%%%%%%%%%%%%%%%%%
  | Tev_Qev_31_75 = ...
  | [
  | 5,15.965       ;
  | 5.1,15.789     ;
  | 5.2,15.794     ;
  | 5.3,15.888     ;
  | 5.4,16.011     ;
  | 5.5,16.275     ;
  | 5.6,16.539     ;
  | 5.7,16.634     ;
  | 5.8,16.57      ;
  | 5.9,16.506     ;
  | 6,16.442       ;
  | 6.1,16.418     ;
  | 6.2,16.401     ;
  | 6.3,16.384     ;
  | 6.4,16.367     ;
  | 6.5,16.35      ;
  | 6.6,16.333     ;
  | 6.7,16.317     ;
  | 6.8,16.652     ;
  | 6.9,17.004     ;
  | 7,17.128       ;
  | 7.1,17.117     ;
  | 7.2,17.106     ;
  | 7.3,17.095     ;
  | 7.4,17.084     ;
  | 7.5,17.073     ;
  | 7.6,17.062     ;
  | 7.7,17.051     ;
  | 7.8,17.04      ;
  | 7.9,17.029     ;
  | 8,17.018       ;
  | 8.1,17.006     ;
  | 8.2,16.994     ;
  | 8.3,16.982     ;
  | 8.4,16.97      ;
  | 8.5,16.959     ;
  | 8.6,16.947     ;
  | 8.7,16.935     ;
  | 8.8,16.923     ;
  | 8.9,16.911     ;
  | 9,16.901       ;
  | 9.1,16.901     ;
  | 9.2,16.901     ;
  | 9.3,16.901     ;
  | 9.4,16.901     ;
  | 9.5,16.901     ;
  | 9.6,16.901     ;
  | 9.7,16.901     ;
  | 9.8,16.901     ;
  | 9.9,16.901     ;
  | 10,16.901      ;
  | 10.1,16.901    ;
  | 10.2,16.901    ;
  | 10.3,16.901    ;
  | 10.4,16.901    ;
  | 10.5,16.901    ;
  | 10.6,16.901    ;
  | 10.7,16.901    ;
  | 10.8,16.901    ;
  | 10.9,16.901    ;
  | 11,16.901      ;
  | 11.1,16.901    ;
  | 11.2,16.901    ;
  | 11.3,16.901    ;
  | 11.4,16.901    ;
  | 11.5,16.901    ;
  | 11.6,16.901    ;
  | 11.7,16.901    ;
  | 11.8,16.901    ;
  | 11.9,16.901    ;
  | 12.0,16.901
  | ];
  | 
  | Tev_Qev_31_80 = ...
  | [
  | 5,23.567       ;
  | 5.1,23.902     ;
  | 5.2,24.17      ;
  | 5.3,24.239     ;
  | 5.4,24.309     ;
  | 5.5,24.379     ;
  | 5.6,24.448     ;
  | 5.7,24.518     ;
  | 5.8,24.588     ;
  | 5.9,24.657     ;
  | 6,24.727       ;
  | 6.1,24.879     ;
  | 6.2,25.044     ;
  | 6.3,25.21      ;
  | 6.4,25.375     ;
  | 6.5,25.541     ;
  | 6.6,25.682     ;
  | 6.7,25.729     ;
  | 6.8,25.776     ;
  | 6.9,25.895     ;
  | 7,26.03        ;
  | 7.1,26.085     ;
  | 7.2,26.139     ;
  | 7.3,26.507     ;
  | 7.4,26.886     ;
  | 7.5,27.003     ;
  | 7.6,27.057     ;
  | 7.7,27.349     ;
  | 7.8,27.395     ;
  | 7.9,27.356     ;
  | 8,27.317       ;
  | 8.1,27.33      ;
  | 8.2,27.354     ;
  | 8.3,27.378     ;
  | 8.4,27.402     ;
  | 8.5,27.426     ;
  | 8.6,27.45      ;
  | 8.7,27.474     ;
  | 8.8,27.498     ;
  | 8.9,27.522     ;
  | 9,27.544       ;
  | 9.1,27.548     ;
  | 9.2,27.552     ;
  | 9.3,27.556     ;
  | 9.4,27.56      ;
  | 9.5,27.564     ;
  | 9.6,27.568     ;
  | 9.7,27.572     ;
  | 9.8,27.576     ;
  | 9.9,27.58      ;
  | 10,27.583      ;
  | 10.1,27.587    ;
  | 10.2,27.591    ;
  | 10.3,27.595    ;
  | 10.4,27.599    ;
  | 10.5,27.603    ;
  | 10.6,27.607    ;
  | 10.7,27.611    ;
  | 10.8,27.615    ;
  | 10.9,27.619    ;
  | 11,27.623      ;
  | 11.1,27.627    ;
  | 11.2,27.63     ;
  | 11.3,27.634    ;
  | 11.4,27.638    ;
  | 11.5,27.642    ;
  | 11.6,27.646    ;
  | 11.7,27.65     ;
  | 11.8,27.654    ;
  | 11.9,27.658    ;
  | 12.0,27.658
  | ];
  | 
  | Tev_Qev_31_85 = ...
  | [
  | 5,26.725       ;
  | 5.1,26.901     ;
  | 5.2,27.094     ;
  | 5.3,27.295     ;
  | 5.4,27.496     ;
  | 5.5,27.693     ;
  | 5.6,27.871     ;
  | 5.7,28.05      ;
  | 5.8,28.229     ;
  | 5.9,28.407     ;
  | 6,28.586       ;
  | 6.1,28.747     ;
  | 6.2,28.907     ;
  | 6.3,29.067     ;
  | 6.4,29.324     ;
  | 6.5,29.831     ;
  | 6.6,30.225     ;
  | 6.7,30.183     ;
  | 6.8,30.14      ;
  | 6.9,30.247     ;
  | 7,30.528       ;
  | 7.1,30.809     ;
  | 7.2,31.262     ;
  | 7.3,31.721     ;
  | 7.4,32.18      ;
  | 7.5,32.573     ;
  | 7.6,32.627     ;
  | 7.7,33.492     ;
  | 7.8,33.518     ;
  | 7.9,33.527     ;
  | 8,33.536       ;
  | 8.1,33.545     ;
  | 8.2,33.554     ;
  | 8.3,33.563     ;
  | 8.4,33.572     ;
  | 8.5,33.581     ;
  | 8.6,33.59      ;
  | 8.7,33.599     ;
  | 8.8,33.608     ;
  | 8.9,33.618     ;
  | 9,33.611       ;
  | 9.1,33.455     ;
  | 9.2,33.298     ;
  | 9.3,33.166     ;
  | 9.4,33.038     ;
  | 9.5,32.921     ;
  | 9.6,32.891     ;
  | 9.7,32.861     ;
  | 9.8,32.831     ;
  | 9.9,32.775     ;
  | 10,32.614      ;
  | 10.1,32.453    ;
  | 10.2,32.347    ;
  | 10.3,32.374    ;
  | 10.4,32.402    ;
  | 10.5,32.429    ;
  | 10.6,32.456    ;
  | 10.7,32.484    ;
  | 10.8,32.511    ;
  | 10.9,32.538    ;
  | 11,32.566      ;
  | 11.1,32.573    ;
  | 11.2,32.573    ;
  | 11.3,32.573    ;
  | 11.4,32.573    ;
  | 11.5,32.573    ;
  | 11.6,32.573    ;
  | 11.7,32.573    ;
  | 11.8,32.573    ;
  | 11.9,32.573    ;
  | 12.0,32.573
  | ];
  | 
  | Tev_Qev_31_88 = ...
  | [
  | 5,30.958      ;
  | 5.1,31.221    ;
  | 5.2,31.401    ;
  | 5.3,31.552    ;
  | 5.4,31.704    ;
  | 5.5,31.855    ;
  | 5.6,32.007    ;
  | 5.7,32.193    ;
  | 5.8,32.445    ;
  | 5.9,32.697    ;
  | 6,32.949      ;
  | 6.1,33.201    ;
  | 6.2,33.453    ;
  | 6.3,33.646    ;
  | 6.4,33.822    ;
  | 6.5,33.997    ;
  | 6.6,34.173    ;
  | 6.7,34.349    ;
  | 6.8,34.525    ;
  | 6.9,34.701    ;
  | 7,34.893      ;
  | 7.1,35.104    ;
  | 7.2,35.11     ;
  | 7.3,35.064    ;
  | 7.4,35.239    ;
  | 7.5,35.731    ;
  | 7.6,35.731    ;
  | 7.7,35.731    ;
  | 7.8,35.731    ;
  | 7.9,35.731    ;
  | 8,35.731      ;
  | 8.1,35.731    ;
  | 8.2,35.731    ;
  | 8.3,35.767    ;
  | 8.4,35.917    ;
  | 8.5,36.066    ;
  | 8.6,36.215    ;
  | 8.7,36.364    ;
  | 8.8,36.514    ;
  | 8.9,36.55     ;
  | 9,36.55       ;
  | 9.1,36.55     ;
  | 9.2,36.55     ;
  | 9.3,36.55     ;
  | 9.4,36.55     ;
  | 9.5,36.55     ;
  | 9.6,36.55     ;
  | 9.7,36.55     ;
  | 9.8,36.55     ;
  | 9.9,36.648    ;
  | 10,36.833     ;
  | 10.1,37.018   ;
  | 10.2,37.135   ;
  | 10.3,37.135   ;
  | 10.4,37.135   ;
  | 10.5,37.135   ;
  | 10.6,37.135   ;
  | 10.7,37.135   ;
  | 10.8,37.135   ;
  | 10.9,37.135   ;
  | 11,37.135     ;
  | 11.1,37.135   ;
  | 11.2,37.135   ;
  | 11.3,37.135   ;
  | 11.4,37.135   ;
  | 11.5,37.135   ;
  | 11.6,37.135   ;
  | 11.7,37.135   ;
  | 11.8,37.135   ;
  | 11.9,37.135   ;
  | 12.0,37.135
  | ];
  | 
  | Tev_Qev_31_95 = ...
  | [
  | 5,31.659       ;
  | 5.1,31.923     ;
  | 5.2,32.5       ;
  | 5.3,33.179     ;
  | 5.4,33.725     ;
  | 5.5,34.014     ;
  | 5.6,34.304     ;
  | 5.7,34.626     ;
  | 5.8,34.977     ;
  | 5.9,35.329     ;
  | 6,35.681       ;
  | 6.1,36.133     ;
  | 6.2,36.602     ;
  | 6.3,37.071     ;
  | 6.4,37.54      ;
  | 6.5,38.009     ;
  | 6.6,38.364     ;
  | 6.7,38.701     ;
  | 6.8,39.039     ;
  | 6.9,39.377     ;
  | 7,39.843       ;
  | 7.1,40.345     ;
  | 7.2,40.741     ;
  | 7.3,41.136     ;
  | 7.4,41.444     ;
  | 7.5,41.652     ;
  | 7.6,41.996     ;
  | 7.7,42.248     ;
  | 7.8,42.198     ;
  | 7.9,42.286     ;
  | 8,42.67        ;
  | 8.1,43.053     ;
  | 8.2,43.2       ;
  | 8.3,43.172     ;
  | 8.4,43.144     ;
  | 8.5,43.116     ;
  | 8.6,43.155     ;
  | 8.7,43.288     ;
  | 8.8,43.421     ;
  | 8.9,43.554     ;
  | 9,43.687       ;
  | 9.1,43.82      ;
  | 9.2,43.953     ;
  | 9.3,44.086     ;
  | 9.4,44.218     ;
  | 9.5,44.351     ;
  | 9.6,44.484     ;
  | 9.7,44.475     ;
  | 9.8,44.442     ;
  | 9.9,44.409     ;
  | 10,44.377      ;
  | 10.1,44.344    ;
  | 10.2,44.311    ;
  | 10.3,44.278    ;
  | 10.4,44.706    ;
  | 10.5,45.088    ;
  | 10.6,45.088    ;
  | 10.7,45.088    ;
  | 10.8,45.088    ;
  | 10.9,45.088    ;
  | 11,45.088      ;
  | 11.1,45.088    ;
  | 11.2,45.088    ;
  | 11.3,45.088    ;
  | 11.4,45.088    ;
  | 11.5,45.088    ;
  | 11.6,45.088    ;
  | 11.7,45.088    ;
  | 11.8,45.088    ;
  | 11.9,45.088    ;
  | 12.0,45.088
  | ];
  | 
  | Tev_COP_31_75 = ...
  | [
  | 5,0.643        ;
  | 5.1,0.647      ;
  | 5.2,0.652      ;
  | 5.3,0.657      ;
  | 5.4,0.663      ;
  | 5.5,0.67       ;
  | 5.6,0.677      ;
  | 5.7,0.682      ;
  | 5.8,0.685      ;
  | 5.9,0.689      ;
  | 6,0.693        ;
  | 6.1,0.697      ;
  | 6.2,0.703      ;
  | 6.3,0.71       ;
  | 6.4,0.717      ;
  | 6.5,0.723      ;
  | 6.6,0.729      ;
  | 6.7,0.734      ;
  | 6.8,0.738      ;
  | 6.9,0.742      ;
  | 7,0.745        ;
  | 7.1,0.748      ;
  | 7.2,0.754      ;
  | 7.3,0.755      ;
  | 7.4,0.755      ;
  | 7.5,0.755      ;
  | 7.6,0.755      ;
  | 7.7,0.754      ;
  | 7.8,0.75       ;
  | 7.9,0.748      ;
  | 8,0.748        ;
  | 8.1,0.748      ;
  | 8.2,0.748      ;
  | 8.3,0.748      ;
  | 8.4,0.747      ;
  | 8.5,0.747      ;
  | 8.6,0.747      ;
  | 8.7,0.747      ;
  | 8.8,0.747      ;
  | 8.9,0.747      ;
  | 9,0.747        ;
  | 9.1,0.747      ;
  | 9.2,0.747      ;
  | 9.3,0.747      ;
  | 9.4,0.747      ;
  | 9.5,0.747      ;
  | 9.6,0.747      ;
  | 9.7,0.747      ;
  | 9.8,0.747      ;
  | 9.9,0.747      ;
  | 10,0.747       ;
  | 10.1,0.747     ;
  | 10.2,0.747     ;
  | 10.3,0.747     ;
  | 10.4,0.747     ;
  | 10.5,0.747     ;
  | 10.6,0.747     ;
  | 10.7,0.747     ;
  | 10.8,0.748     ;
  | 10.9,0.748     ;
  | 11,0.748       ;
  | 11.1,0.748     ;
  | 11.2,0.748     ;
  | 11.3,0.748     ;
  | 11.4,0.748     ;
  | 11.5,0.748     ;
  | 11.6,0.748     ;
  | 11.7,0.748     ;
  | 11.8,0.748     ;
  | 11.9,0.748     ;
  | 12.0,0.748
  | ];
  | 
  | Tev_COP_31_80 = ...
  | [
  | 5,0.607       ;
  | 5.1,0.612     ;
  | 5.2,0.619     ;
  | 5.3,0.626     ;
  | 5.4,0.633     ;
  | 5.5,0.64      ;
  | 5.6,0.647     ;
  | 5.7,0.654     ;
  | 5.8,0.66      ;
  | 5.9,0.666     ;
  | 6,0.673       ;
  | 6.1,0.679     ;
  | 6.2,0.685     ;
  | 6.3,0.692     ;
  | 6.4,0.698     ;
  | 6.5,0.704     ;
  | 6.6,0.711     ;
  | 6.7,0.714     ;
  | 6.8,0.718     ;
  | 6.9,0.723     ;
  | 7,0.729       ;
  | 7.1,0.732     ;
  | 7.2,0.734     ;
  | 7.3,0.734     ;
  | 7.4,0.734     ;
  | 7.5,0.735     ;
  | 7.6,0.735     ;
  | 7.7,0.734     ;
  | 7.8,0.728     ;
  | 7.9,0.727     ;
  | 8,0.727       ;
  | 8.1,0.727     ;
  | 8.2,0.727     ;
  | 8.3,0.728     ;
  | 8.4,0.731     ;
  | 8.5,0.734     ;
  | 8.6,0.734     ;
  | 8.7,0.734     ;
  | 8.8,0.734     ;
  | 8.9,0.735     ;
  | 9,0.735       ;
  | 9.1,0.735     ;
  | 9.2,0.735     ;
  | 9.3,0.735     ;
  | 9.4,0.736     ;
  | 9.5,0.736     ;
  | 9.6,0.736     ;
  | 9.7,0.736     ;
  | 9.8,0.736     ;
  | 9.9,0.737     ;
  | 10,0.737      ;
  | 10.1,0.737    ;
  | 10.2,0.737    ;
  | 10.3,0.737    ;
  | 10.4,0.737    ;
  | 10.5,0.737    ;
  | 10.6,0.737    ;
  | 10.7,0.737    ;
  | 10.8,0.737    ;
  | 10.9,0.737    ;
  | 11,0.737      ;
  | 11.1,0.737    ;
  | 11.2,0.737    ;
  | 11.3,0.738    ;
  | 11.4,0.738    ;
  | 11.5,0.738    ;
  | 11.6,0.738    ;
  | 11.7,0.738    ;
  | 11.8,0.738    ;
  | 11.9,0.738    ;
  | 12.0,0.738
  | ];
  | 
  | Tev_COP_31_85 = ...
  | [
  | 5,0.628       ;
  | 5.1,0.635     ;
  | 5.2,0.641     ;
  | 5.3,0.647     ;
  | 5.4,0.652     ;
  | 5.5,0.657     ;
  | 5.6,0.664     ;
  | 5.7,0.671     ;
  | 5.8,0.678     ;
  | 5.9,0.685     ;
  | 6,0.691       ;
  | 6.1,0.695     ;
  | 6.2,0.699     ;
  | 6.3,0.704     ;
  | 6.4,0.708     ;
  | 6.5,0.713     ;
  | 6.6,0.718     ;
  | 6.7,0.726     ;
  | 6.8,0.733     ;
  | 6.9,0.736     ;
  | 7,0.738       ;
  | 7.1,0.74      ;
  | 7.2,0.744     ;
  | 7.3,0.746     ;
  | 7.4,0.746     ;
  | 7.5,0.745     ;
  | 7.6,0.74      ;
  | 7.7,0.739     ;
  | 7.8,0.739     ;
  | 7.9,0.739     ;
  | 8,0.739       ;
  | 8.1,0.739     ;
  | 8.2,0.739     ;
  | 8.3,0.739     ;
  | 8.4,0.739     ;
  | 8.5,0.739     ;
  | 8.6,0.739     ;
  | 8.7,0.739     ;
  | 8.8,0.739     ;
  | 8.9,0.739     ;
  | 9,0.739       ;
  | 9.1,0.739     ;
  | 9.2,0.739     ;
  | 9.3,0.739     ;
  | 9.4,0.739     ;
  | 9.5,0.739     ;
  | 9.6,0.739     ;
  | 9.7,0.739     ;
  | 9.8,0.739     ;
  | 9.9,0.739     ;
  | 10,0.739      ;
  | 10.1,0.739    ;
  | 10.2,0.739    ;
  | 10.3,0.739    ;
  | 10.4,0.739    ;
  | 10.5,0.739    ;
  | 10.6,0.739    ;
  | 10.7,0.739    ;
  | 10.8,0.739    ;
  | 10.9,0.739    ;
  | 11,0.739      ;
  | 11.1,0.739    ;
  | 11.2,0.739    ;
  | 11.3,0.739    ;
  | 11.4,0.739    ;
  | 11.5,0.739    ;
  | 11.6,0.739    ;
  | 11.7,0.739    ;
  | 11.8,0.739    ;
  | 11.9,0.739    ;
  | 12.0,0.739
  | ];
  | 
  | Tev_COP_31_88 = ...
  | [
  | 5,0.59        ;
  | 5.1,0.599     ;
  | 5.2,0.606     ;
  | 5.3,0.614     ;
  | 5.4,0.619     ;
  | 5.5,0.624     ;
  | 5.6,0.628     ;
  | 5.7,0.634     ;
  | 5.8,0.64      ;
  | 5.9,0.646     ;
  | 6,0.652       ;
  | 6.1,0.659     ;
  | 6.2,0.666     ;
  | 6.3,0.673     ;
  | 6.4,0.679     ;
  | 6.5,0.687     ;
  | 6.6,0.695     ;
  | 6.7,0.703     ;
  | 6.8,0.707     ;
  | 6.9,0.712     ;
  | 7,0.714       ;
  | 7.1,0.718     ;
  | 7.2,0.727     ;
  | 7.3,0.729     ;
  | 7.4,0.729     ;
  | 7.5,0.729     ;
  | 7.6,0.729     ;
  | 7.7,0.729     ;
  | 7.8,0.729     ;
  | 7.9,0.729     ;
  | 8,0.729       ;
  | 8.1,0.729     ;
  | 8.2,0.729     ;
  | 8.3,0.729     ;
  | 8.4,0.729     ;
  | 8.5,0.729     ;
  | 8.6,0.729     ;
  | 8.7,0.729     ;
  | 8.8,0.729     ;
  | 8.9,0.729     ;
  | 9,0.729       ;
  | 9.1,0.729     ;
  | 9.2,0.729     ;
  | 9.3,0.729     ;
  | 9.4,0.729     ;
  | 9.5,0.729     ;
  | 9.6,0.729     ;
  | 9.7,0.729     ;
  | 9.8,0.729     ;
  | 9.9,0.729     ;
  | 10,0.729      ;
  | 10.1,0.729    ;
  | 10.2,0.729    ;
  | 10.3,0.729    ;
  | 10.4,0.729    ;
  | 10.5,0.729    ;
  | 10.6,0.729    ;
  | 10.7,0.729    ;
  | 10.8,0.729    ;
  | 10.9,0.729    ;
  | 11,0.729      ;
  | 11.1,0.729    ;
  | 11.2,0.729    ;
  | 11.3,0.729    ;
  | 11.4,0.729    ;
  | 11.5,0.729    ;
  | 11.6,0.729    ;
  | 11.7,0.729    ;
  | 11.8,0.729    ;
  | 11.9,0.729    ;
  | 12.0,0.729
  | ];
  | 
  | Tev_COP_31_95 = ...
  | [
  | 5,0.513      ;
  | 5.1,0.519    ;
  | 5.2,0.526    ;
  | 5.3,0.534    ;
  | 5.4,0.541    ;
  | 5.5,0.548    ;
  | 5.6,0.554    ;
  | 5.7,0.56     ;
  | 5.8,0.565    ;
  | 5.9,0.571    ;
  | 6,0.578      ;
  | 6.1,0.584    ;
  | 6.2,0.59     ;
  | 6.3,0.594    ;
  | 6.4,0.599    ;
  | 6.5,0.607    ;
  | 6.6,0.615    ;
  | 6.7,0.622    ;
  | 6.8,0.626    ;
  | 6.9,0.63     ;
  | 7,0.634      ;
  | 7.1,0.64     ;
  | 7.2,0.646    ;
  | 7.3,0.658    ;
  | 7.4,0.666    ;
  | 7.5,0.671    ;
  | 7.6,0.677    ;
  | 7.7,0.682    ;
  | 7.8,0.686    ;
  | 7.9,0.687    ;
  | 8,0.687      ;
  | 8.1,0.686    ;
  | 8.2,0.692    ;
  | 8.3,0.696    ;
  | 8.4,0.696    ;
  | 8.5,0.696    ;
  | 8.6,0.696    ;
  | 8.7,0.696    ;
  | 8.8,0.695    ;
  | 8.9,0.695    ;
  | 9,0.695      ;
  | 9.1,0.695    ;
  | 9.2,0.695    ;
  | 9.3,0.695    ;
  | 9.4,0.696    ;
  | 9.5,0.698    ;
  | 9.6,0.7      ;
  | 9.7,0.7      ;
  | 9.8,0.7      ;
  | 9.9,0.7      ;
  | 10,0.7       ;
  | 10.1,0.7     ;
  | 10.2,0.7     ;
  | 10.3,0.7     ;
  | 10.4,0.7     ;
  | 10.5,0.7     ;
  | 10.6,0.7     ;
  | 10.7,0.7     ;
  | 10.8,0.7     ;
  | 10.9,0.7     ;
  | 11,0.7       ;
  | 11.1,0.7     ;
  | 11.2,0.7     ;
  | 11.3,0.7     ;
  | 11.4,0.7     ;
  | 11.5,0.7     ;
  | 11.6,0.7     ;
  | 11.7,0.7     ;
  | 11.8,0.7     ;
  | 11.9,0.7     ;
  | 12.0,0.7
  | ];
  | 
  | 
  | % 32 ºC
  | %%%%%%%%%%%%%%%%%%%%%%%%%%%%%%%%%%%%%%%%%%%%%%%%%%
  | Tev_Qev_32_75 = ...
  | [
  | 5,10.93       ;
  | 5.1,10.914    ;
  | 5.2,10.897    ;
  | 5.3,10.881    ;
  | 5.4,10.865    ;
  | 5.5,10.848    ;
  | 5.6,10.832    ;
  | 5.7,10.815    ;
  | 5.8,10.799    ;
  | 5.9,10.783    ;
  | 6,10.766      ;
  | 6.1,10.75     ;
  | 6.2,10.734    ;
  | 6.3,10.717    ;
  | 6.4,10.701    ;
  | 6.5,10.981    ;
  | 6.6,11.329    ;
  | 6.7,11.508    ;
  | 6.8,11.499    ;
  | 6.9,11.49     ;
  | 7,11.481      ;
  | 7.1,11.473    ;
  | 7.2,11.464    ;
  | 7.3,11.455    ;
  | 7.4,11.447    ;
  | 7.5,11.438    ;
  | 7.6,11.429    ;
  | 7.7,11.421    ;
  | 7.8,11.412    ;
  | 7.9,11.403    ;
  | 8,11.395      ;
  | 8.1,11.395    ;
  | 8.2,11.395    ;
  | 8.3,11.395    ;
  | 8.4,11.395    ;
  | 8.5,11.395    ;
  | 8.6,11.395    ;
  | 8.7,11.395    ;
  | 8.8,11.395    ;
  | 8.9,11.395    ;
  | 9,11.395      ;
  | 9.1,11.395    ;
  | 9.2,11.395    ;
  | 9.3,11.395    ;
  | 9.4,11.395    ;
  | 9.5,11.395    ;
  | 9.6,11.395    ;
  | 9.7,11.395    ;
  | 9.8,11.395    ;
  | 9.9,11.395    ;
  | 10,11.395     ;
  | 10.1,11.395   ;
  | 10.2,11.395   ;
  | 10.3,11.395   ;
  | 10.4,11.395   ;
  | 10.5,11.395   ;
  | 10.6,11.395   ;
  | 10.7,11.395   ;
  | 10.8,11.395   ;
  | 10.9,11.395   ;
  | 11,11.395     ;
  | 11.1,11.395   ;
  | 11.2,11.395   ;
  | 11.3,11.395   ;
  | 11.4,11.395   ;
  | 11.5,11.395   ;
  | 11.6,11.395   ;
  | 11.7,11.395   ;
  | 11.8,11.395   ;
  | 11.9,11.395   ;
  | 12.0,11.395
  | ];
  | 
  | Tev_Qev_32_80 = ...
  | [
  | 5,18.739      ;
  | 5.1,18.967    ;
  | 5.2,19.18     ;
  | 5.3,19.393    ;
  | 5.4,19.607    ;
  | 5.5,19.82     ;
  | 5.6,20.033    ;
  | 5.7,20.135    ;
  | 5.8,20.165    ;
  | 5.9,20.196    ;
  | 6,20.226      ;
  | 6.1,20.358    ;
  | 6.2,20.516    ;
  | 6.3,20.675    ;
  | 6.4,20.814    ;
  | 6.5,20.814    ;
  | 6.6,20.814    ;
  | 6.7,20.814    ;
  | 6.8,20.814    ;
  | 6.9,20.814    ;
  | 7,21.014      ;
  | 7.1,21.353    ;
  | 7.2,21.407    ;
  | 7.3,21.419    ;
  | 7.4,21.432    ;
  | 7.5,21.445    ;
  | 7.6,21.458    ;
  | 7.7,21.471    ;
  | 7.8,21.484    ;
  | 7.9,21.497    ;
  | 8,21.509      ;
  | 8.1,21.509    ;
  | 8.2,21.506    ;
  | 8.3,21.503    ;
  | 8.4,21.5      ;
  | 8.5,21.497    ;
  | 8.6,21.494    ;
  | 8.7,21.492    ;
  | 8.8,21.489    ;
  | 8.9,21.486    ;
  | 9,21.483      ;
  | 9.1,21.48     ;
  | 9.2,21.477    ;
  | 9.3,21.474    ;
  | 9.4,21.471    ;
  | 9.5,21.468    ;
  | 9.6,21.465    ;
  | 9.7,21.462    ;
  | 9.8,21.459    ;
  | 9.9,21.456    ;
  | 10,21.453     ;
  | 10.1,21.45    ;
  | 10.2,21.448   ;
  | 10.3,21.445   ;
  | 10.4,21.442   ;
  | 10.5,21.439   ;
  | 10.6,21.436   ;
  | 10.7,21.433   ;
  | 10.8,21.43    ;
  | 10.9,21.427   ;
  | 11,21.424     ;
  | 11.1,21.421   ;
  | 11.2,21.418   ;
  | 11.3,21.415   ;
  | 11.4,21.412   ;
  | 11.5,21.409   ;
  | 11.6,21.406   ;
  | 11.7,21.403   ;
  | 11.8,21.401   ;
  | 11.9,21.398   ;
  | 12.0,21.398
  | ];
  | 
  | Tev_Qev_32_85 = ...
  | [
  | 5,21.217      ;
  | 5.1,21.913    ;
  | 5.2,22.359    ;
  | 5.3,22.78     ;
  | 5.4,23.201    ;
  | 5.5,23.57     ;
  | 5.6,23.932    ;
  | 5.7,24.307    ;
  | 5.8,24.713    ;
  | 5.9,25.12     ;
  | 6,25.527      ;
  | 6.1,25.91     ;
  | 6.2,26.289    ;
  | 6.3,26.668    ;
  | 6.4,27.048    ;
  | 6.5,27.433    ;
  | 6.6,27.833    ;
  | 6.7,28.234    ;
  | 6.8,28.635    ;
  | 6.9,29.036    ;
  | 7,29.428      ;
  | 7.1,29.649    ;
  | 7.2,29.87     ;
  | 7.3,30.001    ;
  | 7.4,30.181    ;
  | 7.5,30.631    ;
  | 7.6,30.199    ;
  | 7.7,30        ;
  | 7.8,30        ;
  | 7.9,30        ;
  | 8,30          ;
  | 8.1,30        ;
  | 8.2,30        ;
  | 8.3,30.194    ;
  | 8.4,30.492    ;
  | 8.5,30.567    ;
  | 8.6,30.547    ;
  | 8.7,30.526    ;
  | 8.8,30.506    ;
  | 8.9,30.485    ;
  | 9,30.466      ;
  | 9.1,30.532    ;
  | 9.2,30.597    ;
  | 9.3,30.663    ;
  | 9.4,30.729    ;
  | 9.5,30.795    ;
  | 9.6,30.814    ;
  | 9.7,30.814    ;
  | 9.8,30.814    ;
  | 9.9,30.814    ;
  | 10,30.814     ;
  | 10.1,30.814   ;
  | 10.2,30.814   ;
  | 10.3,30.814   ;
  | 10.4,30.814   ;
  | 10.5,30.814   ;
  | 10.6,30.814   ;
  | 10.7,30.814   ;
  | 10.8,30.814   ;
  | 10.9,30.814   ;
  | 11,30.815     ;
  | 11.1,30.826   ;
  | 11.2,30.838   ;
  | 11.3,30.85    ;
  | 11.4,30.862   ;
  | 11.5,30.874   ;
  | 11.6,30.886   ;
  | 11.7,30.897   ;
  | 11.8,30.909   ;
  | 11.9,30.921   ;
  | 12.0,30.921
  | ];
  | 
  | Tev_Qev_32_88 = ...
  | [
  | 5,26.279       ;
  | 5.1,26.294     ;
  | 5.2,26.52      ;
  | 5.3,26.746     ;
  | 5.4,27.038     ;
  | 5.5,27.564     ;
  | 5.6,28.09      ;
  | 5.7,28.501     ;
  | 5.8,28.858     ;
  | 5.9,29.215     ;
  | 6,29.572       ;
  | 6.1,29.929     ;
  | 6.2,30.281     ;
  | 6.3,30.601     ;
  | 6.4,30.92      ;
  | 6.5,31.126     ;
  | 6.6,31.327     ;
  | 6.7,31.542     ;
  | 6.8,31.895     ;
  | 6.9,32.248     ;
  | 7,32.592       ;
  | 7.1,32.872     ;
  | 7.2,33.152     ;
  | 7.3,33.256     ;
  | 7.4,33.445     ;
  | 7.5,33.856     ;
  | 7.6,34.181     ;
  | 7.7,34.154     ;
  | 7.8,34.126     ;
  | 7.9,34.099     ;
  | 8,34.072       ;
  | 8.1,34.264     ;
  | 8.2,34.477     ;
  | 8.3,34.58      ;
  | 8.4,34.642     ;
  | 8.5,34.806     ;
  | 8.6,34.987     ;
  | 8.7,35.129     ;
  | 8.8,35.173     ;
  | 8.9,35.217     ;
  | 9,35.326       ;
  | 9.1,35.473     ;
  | 9.2,35.62      ;
  | 9.3,35.767     ;
  | 9.4,35.914     ;
  | 9.5,36.047     ;
  | 9.6,36.047     ;
  | 9.7,36.047     ;
  | 9.8,36.047     ;
  | 9.9,36.047     ;
  | 10,36.053      ;
  | 10.1,36.087    ;
  | 10.2,36.122    ;
  | 10.3,36.156    ;
  | 10.4,36.191    ;
  | 10.5,36.225    ;
  | 10.6,36.26     ;
  | 10.7,36.294    ;
  | 10.8,36.328    ;
  | 10.9,36.363    ;
  | 11,36.396      ;
  | 11.1,36.408    ;
  | 11.2,36.419    ;
  | 11.3,36.431    ;
  | 11.4,36.443    ;
  | 11.5,36.454    ;
  | 11.6,36.466    ;
  | 11.7,36.478    ;
  | 11.8,36.489    ;
  | 11.9,36.501    ;
  | 12.0,36.501
  | ];
  | 
  | Tev_Qev_32_95 = ...
  | [
  | 5,31.532      ;
  | 5.1,31.8      ;
  | 5.2,32.067    ;
  | 5.3,32.334    ;
  | 5.4,32.601    ;
  | 5.5,32.868    ;
  | 5.6,33.266    ;
  | 5.7,33.685    ;
  | 5.8,34.105    ;
  | 5.9,34.524    ;
  | 6,34.944      ;
  | 6.1,35.332    ;
  | 6.2,35.716    ;
  | 6.3,36.099    ;
  | 6.4,36.483    ;
  | 6.5,36.867    ;
  | 6.6,37.25     ;
  | 6.7,37.634    ;
  | 6.8,38.017    ;
  | 6.9,38.252    ;
  | 7,38.833      ;
  | 7.1,39.392    ;
  | 7.2,39.718    ;
  | 7.3,39.801    ;
  | 7.4,39.735    ;
  | 7.5,40.303    ;
  | 7.6,40.581    ;
  | 7.7,40.777    ;
  | 7.8,41.163    ;
  | 7.9,41.163    ;
  | 8,41.163      ;
  | 8.1,41.321    ;
  | 8.2,41.511    ;
  | 8.3,41.701    ;
  | 8.4,41.89     ;
  | 8.5,41.977    ;
  | 8.6,41.977    ;
  | 8.7,42.005    ;
  | 8.8,42.223    ;
  | 8.9,42.442    ;
  | 9,42.66       ;
  | 9.1,42.695    ;
  | 9.2,42.717    ;
  | 9.3,42.74     ;
  | 9.4,42.762    ;
  | 9.5,42.784    ;
  | 9.6,42.861    ;
  | 9.7,42.961    ;
  | 9.8,43.116    ;
  | 9.9,43.364    ;
  | 10,43.607     ;
  | 10.1,43.677   ;
  | 10.2,43.747   ;
  | 10.3,43.817   ;
  | 10.4,43.887   ;
  | 10.5,43.949   ;
  | 10.6,43.858   ;
  | 10.7,43.766   ;
  | 10.8,43.674   ;
  | 10.9,43.582   ;
  | 11,43.49      ;
  | 11.1,43.465   ;
  | 11.2,43.442   ;
  | 11.3,43.418   ;
  | 11.4,43.394   ;
  | 11.5,43.371   ;
  | 11.6,43.347   ;
  | 11.7,43.323   ;
  | 11.8,43.299   ;
  | 11.9,43.276   ;
  | 12.0,43.276
  | ];
  | 
  | Tev_COP_32_75 = ...
  | [
  | 5.0,0.506     ;
  | 5.1,0.507     ;
  | 5.2,0.516     ;
  | 5.3,0.522     ;
  | 5.4,0.527     ;
  | 5.5,0.533     ;
  | 5.6,0.539     ;
  | 5.7,0.545     ;
  | 5.8,0.551     ;
  | 5.9,0.557     ;
  | 6,0.564       ;
  | 6.1,0.571     ;
  | 6.2,0.58      ;
  | 6.3,0.589     ;
  | 6.4,0.597     ;
  | 6.5,0.601     ;
  | 6.6,0.605     ;
  | 6.7,0.61      ;
  | 6.8,0.615     ;
  | 6.9,0.62      ;
  | 7,0.625       ;
  | 7.1,0.63      ;
  | 7.2,0.636     ;
  | 7.3,0.637     ;
  | 7.4,0.637     ;
  | 7.5,0.636     ;
  | 7.6,0.636     ;
  | 7.7,0.636     ;
  | 7.8,0.632     ;
  | 7.9,0.63      ;
  | 8,0.63        ;
  | 8.1,0.63      ;
  | 8.2,0.63      ;
  | 8.3,0.63      ;
  | 8.4,0.63      ;
  | 8.5,0.63      ;
  | 8.6,0.63      ;
  | 8.7,0.63      ;
  | 8.8,0.63      ;
  | 8.9,0.63      ;
  | 9,0.63        ;
  | 9.1,0.63      ;
  | 9.2,0.63      ;
  | 9.3,0.63      ;
  | 9.4,0.63      ;
  | 9.5,0.63      ;
  | 9.6,0.63      ;
  | 9.7,0.63      ;
  | 9.8,0.63      ;
  | 9.9,0.63      ;
  | 10,0.629      ;
  | 10.1,0.629    ;
  | 10.2,0.629    ;
  | 10.3,0.629    ;
  | 10.4,0.629    ;
  | 10.5,0.629    ;
  | 10.6,0.629    ;
  | 10.7,0.629    ;
  | 10.8,0.629    ;
  | 10.9,0.629    ;
  | 11,0.629      ;
  | 11.1,0.629    ;
  | 11.2,0.629    ;
  | 11.3,0.629    ;
  | 11.4,0.629    ;
  | 11.5,0.629    ;
  | 11.6,0.629    ;
  | 11.7,0.629    ;
  | 11.8,0.629    ;
  | 11.9,0.629    ;
  | 12.0,0.629
  | ];
  | 
  | Tev_COP_32_80 = ...
  | [
  | 5,0.572       ;
  | 5.1,0.576     ;
  | 5.2,0.582     ;
  | 5.3,0.589     ;
  | 5.4,0.595     ;
  | 5.5,0.602     ;
  | 5.6,0.609     ;
  | 5.7,0.616     ;
  | 5.8,0.623     ;
  | 5.9,0.631     ;
  | 6,0.638       ;
  | 6.1,0.645     ;
  | 6.2,0.652     ;
  | 6.3,0.66      ;
  | 6.4,0.667     ;
  | 6.5,0.674     ;
  | 6.6,0.682     ;
  | 6.7,0.688     ;
  | 6.8,0.693     ;
  | 6.9,0.698     ;
  | 7,0.707       ;
  | 7.1,0.712     ;
  | 7.2,0.718     ;
  | 7.3,0.718     ;
  | 7.4,0.718     ;
  | 7.5,0.718     ;
  | 7.6,0.713     ;
  | 7.7,0.712     ;
  | 7.8,0.711     ;
  | 7.9,0.71      ;
  | 8,0.71        ;
  | 8.1,0.71      ;
  | 8.2,0.71      ;
  | 8.3,0.71      ;
  | 8.4,0.71      ;
  | 8.5,0.71      ;
  | 8.6,0.71      ;
  | 8.7,0.71      ;
  | 8.8,0.711     ;
  | 8.9,0.711     ;
  | 9,0.711       ;
  | 9.1,0.711     ;
  | 9.2,0.711     ;
  | 9.3,0.711     ;
  | 9.4,0.711     ;
  | 9.5,0.711     ;
  | 9.6,0.711     ;
  | 9.7,0.711     ;
  | 9.8,0.711     ;
  | 9.9,0.711     ;
  | 10,0.711      ;
  | 10.1,0.711    ;
  | 10.2,0.711    ;
  | 10.3,0.711    ;
  | 10.4,0.711    ;
  | 10.5,0.711    ;
  | 10.6,0.711    ;
  | 10.7,0.711    ;
  | 10.8,0.711    ;
  | 10.9,0.711    ;
  | 11,0.711      ;
  | 11.1,0.711    ;
  | 11.2,0.711    ;
  | 11.3,0.711    ;
  | 11.4,0.711    ;
  | 11.5,0.711    ;
  | 11.6,0.711    ;
  | 11.7,0.711    ;
  | 11.8,0.711    ;
  | 11.9,0.711    ;
  | 12.0,0.711
  | ];
  | 
  | Tev_COP_32_85 = ...
  | [
  | 5,0.547       ;
  | 5.1,0.553     ;
  | 5.2,0.558     ;
  | 5.3,0.564     ;
  | 5.4,0.572     ;
  | 5.5,0.58      ;
  | 5.6,0.589     ;
  | 5.7,0.598     ;
  | 5.8,0.607     ;
  | 5.9,0.615     ;
  | 6,0.624       ;
  | 6.1,0.632     ;
  | 6.2,0.641     ;
  | 6.3,0.648     ;
  | 6.4,0.655     ;
  | 6.5,0.665     ;
  | 6.6,0.676     ;
  | 6.7,0.684     ;
  | 6.8,0.688     ;
  | 6.9,0.692     ;
  | 7,0.697       ;
  | 7.1,0.703     ;
  | 7.2,0.709     ;
  | 7.3,0.715     ;
  | 7.4,0.72      ;
  | 7.5,0.723     ;
  | 7.6,0.723     ;
  | 7.7,0.717     ;
  | 7.8,0.715     ;
  | 7.9,0.716     ;
  | 8,0.717       ;
  | 8.1,0.717     ;
  | 8.2,0.718     ;
  | 8.3,0.719     ;
  | 8.4,0.721     ;
  | 8.5,0.722     ;
  | 8.6,0.722     ;
  | 8.7,0.722     ;
  | 8.8,0.724     ;
  | 8.9,0.727     ;
  | 9,0.729       ;
  | 9.1,0.729     ;
  | 9.2,0.729     ;
  | 9.3,0.729     ;
  | 9.4,0.729     ;
  | 9.5,0.729     ;
  | 9.6,0.728     ;
  | 9.7,0.728     ;
  | 9.8,0.728     ;
  | 9.9,0.728     ;
  | 10,0.728      ;
  | 10.1,0.728    ;
  | 10.2,0.728    ;
  | 10.3,0.728    ;
  | 10.4,0.728    ;
  | 10.5,0.728    ;
  | 10.6,0.728    ;
  | 10.7,0.728    ;
  | 10.8,0.728    ;
  | 10.9,0.728    ;
  | 11,0.728      ;
  | 11.1,0.728    ;
  | 11.2,0.728    ;
  | 11.3,0.728    ;
  | 11.4,0.728    ;
  | 11.5,0.728    ;
  | 11.6,0.728    ;
  | 11.7,0.728    ;
  | 11.8,0.728    ;
  | 11.9,0.728    ;
  | 12.0,0.728
  | ];
  | 
  | Tev_COP_32_88 = ...
  | [
  | 5,0.523      ;
  | 5.1,0.532    ;
  | 5.2,0.54     ;
  | 5.3,0.548    ;
  | 5.4,0.555    ;
  | 5.5,0.563    ;
  | 5.6,0.572    ;
  | 5.7,0.581    ;
  | 5.8,0.591    ;
  | 5.9,0.6      ;
  | 6,0.609      ;
  | 6.1,0.617    ;
  | 6.2,0.624    ;
  | 6.3,0.633    ;
  | 6.4,0.643    ;
  | 6.5,0.654    ;
  | 6.6,0.665    ;
  | 6.7,0.674    ;
  | 6.8,0.681    ;
  | 6.9,0.687    ;
  | 7,0.694      ;
  | 7.1,0.699    ;
  | 7.2,0.703    ;
  | 7.3,0.709    ;
  | 7.4,0.712    ;
  | 7.5,0.71     ;
  | 7.6,0.71     ;
  | 7.7,0.71     ;
  | 7.8,0.71     ;
  | 7.9,0.71     ;
  | 8,0.71       ;
  | 8.1,0.711    ;
  | 8.2,0.711    ;
  | 8.3,0.711    ;
  | 8.4,0.711    ;
  | 8.5,0.712    ;
  | 8.6,0.712    ;
  | 8.7,0.712    ;
  | 8.8,0.714    ;
  | 8.9,0.717    ;
  | 9,0.718      ;
  | 9.1,0.718    ;
  | 9.2,0.718    ;
  | 9.3,0.718    ;
  | 9.4,0.718    ;
  | 9.5,0.718    ;
  | 9.6,0.718    ;
  | 9.7,0.718    ;
  | 9.8,0.718    ;
  | 9.9,0.718    ;
  | 10,0.718     ;
  | 10.1,0.718   ;
  | 10.2,0.718   ;
  | 10.3,0.718   ;
  | 10.4,0.718   ;
  | 10.5,0.718   ;
  | 10.6,0.718   ;
  | 10.7,0.718   ;
  | 10.8,0.718   ;
  | 10.9,0.718   ;
  | 11,0.718     ;
  | 11.1,0.718   ;
  | 11.2,0.718   ;
  | 11.3,0.718   ;
  | 11.4,0.718   ;
  | 11.5,0.718   ;
  | 11.6,0.718   ;
  | 11.7,0.718   ;
  | 11.8,0.718   ;
  | 11.9,0.718   ;
  | 12.0,0.718
  | ];
  | 
  | Tev_COP_32_95 = ...
  | [
  | 5.0,0.508    ;
  | 5.1,0.509    ;
  | 5.2,0.516    ;
  | 5.3,0.522    ;
  | 5.4,0.528    ;
  | 5.5,0.534    ;
  | 5.6,0.54     ;
  | 5.7,0.546    ;
  | 5.8,0.552    ;
  | 5.9,0.558    ;
  | 6,0.563      ;
  | 6.1,0.569    ;
  | 6.2,0.575    ;
  | 6.3,0.582    ;
  | 6.4,0.589    ;
  | 6.5,0.593    ;
  | 6.6,0.598    ;
  | 6.7,0.602    ;
  | 6.8,0.611    ;
  | 6.9,0.619    ;
  | 7,0.626      ;
  | 7.1,0.633    ;
  | 7.2,0.639    ;
  | 7.3,0.644    ;
  | 7.4,0.648    ;
  | 7.5,0.655    ;
  | 7.6,0.665    ;
  | 7.7,0.671    ;
  | 7.8,0.676    ;
  | 7.9,0.677    ;
  | 8,0.676      ;
  | 8.1,0.679    ;
  | 8.2,0.682    ;
  | 8.3,0.686    ;
  | 8.4,0.689    ;
  | 8.5,0.69     ;
  | 8.6,0.69     ;
  | 8.7,0.69     ;
  | 8.8,0.69     ;
  | 8.9,0.69     ;
  | 9,0.69       ;
  | 9.1,0.69     ;
  | 9.2,0.69     ;
  | 9.3,0.69     ;
  | 9.4,0.69     ;
  | 9.5,0.69     ;
  | 9.6,0.69     ;
  | 9.7,0.69     ;
  | 9.8,0.69     ;
  | 9.9,0.69     ;
  | 10,0.69      ;
  | 10.1,0.69    ;
  | 10.2,0.69    ;
  | 10.3,0.69    ;
  | 10.4,0.69    ;
  | 10.5,0.69    ;
  | 10.6,0.69    ;
  | 10.7,0.69    ;
  | 10.8,0.69    ;
  | 10.9,0.69    ;
  | 11,0.69      ;
  | 11.1,0.69    ;
  | 11.2,0.69    ;
  | 11.3,0.69    ;
  | 11.4,0.69    ;
  | 11.5,0.69    ;
  | 11.6,0.69    ;
  | 11.7,0.69    ;
  | 11.8,0.69    ;
  | 11.9,0.69    ;
  | 12.0,0.69
  | ];
  | 
  | 
  | % 24 ºC
  | Q_Ev(:,1,1) = [Tev_Qev_24_75(:,2); Tev_Qev_24_75(end,2)*ones(length(12.1:0.1:40),1)]; % añado las temperaturas [12.1,..., 40] mantieniendo constante la potencia
  | Q_Ev(:,2,1) = [Tev_Qev_24_80(:,2); Tev_Qev_24_80(end,2)*ones(length(12.1:0.1:40),1)];
  | Q_Ev(:,3,1) = [Tev_Qev_24_85(:,2); Tev_Qev_24_85(end,2)*ones(length(12.1:0.1:40),1)];
  | Q_Ev(:,4,1) = [Tev_Qev_24_88(:,2); Tev_Qev_24_88(end,2)*ones(length(12.1:0.1:40),1)];
  | Q_Ev(:,5,1) = [Tev_Qev_24_95(:,2); Tev_Qev_24_95(end,2)*ones(length(12.1:0.1:40),1)];
  | 
  | COP(:,1,1) = [Tev_COP_24_75(:,2); Tev_COP_24_75(end,2)*ones(length(12.1:0.1:40),1)];
  | COP(:,2,1) = [Tev_COP_24_80(:,2); Tev_COP_24_80(end,2)*ones(length(12.1:0.1:40),1)];
  | COP(:,3,1) = [Tev_COP_24_85(:,2); Tev_COP_24_85(end,2)*ones(length(12.1:0.1:40),1)];
  | COP(:,4,1) = [Tev_COP_24_88(:,2); Tev_COP_24_88(end,2)*ones(length(12.1:0.1:40),1)];
  | COP(:,5,1) = [Tev_COP_24_95(:,2); Tev_COP_24_95(end,2)*ones(length(12.1:0.1:40),1)];
  | 
  | % 29 ºC
  | Q_Ev(:,1,2) = [Tev_Qev_29_75(:,2); Tev_Qev_29_75(end,2)*ones(length(12.1:0.1:40),1)]; % añado las temperaturas [12.1,..., 40] mantieniendo constante la potencia
  | Q_Ev(:,2,2) = [Tev_Qev_29_80(:,2); Tev_Qev_29_80(end,2)*ones(length(12.1:0.1:40),1)];
  | Q_Ev(:,3,2) = [Tev_Qev_29_85(:,2); Tev_Qev_29_85(end,2)*ones(length(12.1:0.1:40),1)];
  | Q_Ev(:,4,2) = [Tev_Qev_29_88(:,2); Tev_Qev_29_88(end,2)*ones(length(12.1:0.1:40),1)];
  | Q_Ev(:,5,2) = [Tev_Qev_29_95(:,2); Tev_Qev_29_95(end,2)*ones(length(12.1:0.1:40),1)];
  | 
  | COP(:,1,2) = [Tev_COP_29_75(:,2); Tev_COP_29_75(end,2)*ones(length(12.1:0.1:40),1)];
  | COP(:,2,2) = [Tev_COP_29_80(:,2); Tev_COP_29_80(end,2)*ones(length(12.1:0.1:40),1)];
  | COP(:,3,2) = [Tev_COP_29_85(:,2); Tev_COP_29_85(end,2)*ones(length(12.1:0.1:40),1)];
  | COP(:,4,2) = [Tev_COP_29_88(:,2); Tev_COP_29_88(end,2)*ones(length(12.1:0.1:40),1)];
  | COP(:,5,2) = [Tev_COP_29_95(:,2); Tev_COP_29_95(end,2)*ones(length(12.1:0.1:40),1)];
  | 
  | % 31 ºC
  | Q_Ev(:,1,3) = [Tev_Qev_31_75(:,2); Tev_Qev_31_75(end,2)*ones(length(12.1:0.1:40),1)]; % añado las temperaturas [12.1,..., 40] mantieniendo constante la potencia
  | Q_Ev(:,2,3) = [Tev_Qev_31_80(:,2); Tev_Qev_31_80(end,2)*ones(length(12.1:0.1:40),1)];
  | Q_Ev(:,3,3) = [Tev_Qev_31_85(:,2); Tev_Qev_31_85(end,2)*ones(length(12.1:0.1:40),1)];
  | Q_Ev(:,4,3) = [Tev_Qev_31_88(:,2); Tev_Qev_31_88(end,2)*ones(length(12.1:0.1:40),1)];
  | Q_Ev(:,5,3) = [Tev_Qev_31_95(:,2); Tev_Qev_31_95(end,2)*ones(length(12.1:0.1:40),1)];
  | 
  | COP(:,1,3) = [Tev_COP_31_75(:,2); Tev_COP_31_75(end,2)*ones(length(12.1:0.1:40),1)];
  | COP(:,2,3) = [Tev_COP_31_80(:,2); Tev_COP_31_80(end,2)*ones(length(12.1:0.1:40),1)];
  | COP(:,3,3) = [Tev_COP_31_85(:,2); Tev_COP_31_85(end,2)*ones(length(12.1:0.1:40),1)];
  | COP(:,4,3) = [Tev_COP_31_88(:,2); Tev_COP_31_88(end,2)*ones(length(12.1:0.1:40),1)];
  | COP(:,5,3) = [Tev_COP_31_95(:,2); Tev_COP_31_95(end,2)*ones(length(12.1:0.1:40),1)];
  | 
  | % 32 ºC
  | Q_Ev(:,1,4) = [Tev_Qev_32_75(:,2); Tev_Qev_31_75(end,2)*ones(length(12.1:0.1:40),1)]; % añado las temperaturas [12.1,..., 40] mantieniendo constante la potencia
  | Q_Ev(:,2,4) = [Tev_Qev_32_80(:,2); Tev_Qev_31_80(end,2)*ones(length(12.1:0.1:40),1)];
  | Q_Ev(:,3,4) = [Tev_Qev_32_85(:,2); Tev_Qev_31_85(end,2)*ones(length(12.1:0.1:40),1)];
  | Q_Ev(:,4,4) = [Tev_Qev_32_88(:,2); Tev_Qev_31_88(end,2)*ones(length(12.1:0.1:40),1)];
  | Q_Ev(:,5,4) = [Tev_Qev_32_95(:,2); Tev_Qev_31_95(end,2)*ones(length(12.1:0.1:40),1)];
  | 
  | COP(:,1,4) = [Tev_COP_32_75(:,2); Tev_COP_32_75(end,2)*ones(length(12.1:0.1:40),1)];
  | COP(:,2,4) = [Tev_COP_32_80(:,2); Tev_COP_32_80(end,2)*ones(length(12.1:0.1:40),1)];
  | COP(:,3,4) = [Tev_COP_32_85(:,2); Tev_COP_32_85(end,2)*ones(length(12.1:0.1:40),1)];
  | COP(:,4,4) = [Tev_COP_32_88(:,2); Tev_COP_32_88(end,2)*ones(length(12.1:0.1:40),1)];
  | COP(:,5,4) = [Tev_COP_32_95(:,2); Tev_COP_32_95(end,2)*ones(length(12.1:0.1:40),1)];
  | 
  | % MESHGRID DE DATA
  | x = [75 80 85 88 95];
  | y = [Tev_Qev_29_75(:,1); (12.1:0.1:40)'];
  | z = [24 29.5 31 32];
  | [Xq1,Yq1,Zq1] = meshgrid(x, y, z);
  | %    [Xq1,Yq1] = meshgrid(x, y);
  | 
  | % INTERPOLACION SUAVE DATA PARA TENER MÁS PUNTOS
  | xi = 75:0.5:95;
  | yi = [Tev_Qev_29_75(:,1); (12.1:0.1:40)'];
  | zi = 24:0.1:32;
  | [Xqevap,Yqevap,Zqevap] = meshgrid(xi, yi, zi);
  | % [Xqevap,Yqevap] = meshgrid(xi, yi);
  | Xcop = Xqevap;
  | Ycop = Yqevap;
  | Zcop = Zqevap;
  | Q_Evap_data = interp3(Xq1,Yq1,Zq1,Q_Ev,Xqevap,Yqevap,Zqevap,'makima');
  | COP_data = interp3(Xq1,Yq1,Zq1,COP,Xcop,Ycop,Zcop,'makima');
values from neighbouring files (symbols this model uses):
  b = 0.5    [Parametros.mat]
  COP = [0 0.070515985287 0.134110087833 0.19134985944 0.242630993683 0.288594392201 0.329807846702 0.366857212964 0.400191394483 0.430176776589 0.45717114527 0.481510123931 ... (8001 elements, 8001x1)]    [ResultadoSimulacion.mat]
  K_ff_eva = 0.87    [Parametros.mat]
  K_ff_tes = 0.63    [Parametros.mat]
  K_ff_tor = 0.9    [Parametros.mat]
  Kd = 4.5    [Parametros.mat]
  Kp = 0.57    [Parametros.mat]
  T_f = 1.214    [Parametros.mat]
  T_t = 7.14    [Parametros.mat]
  Ti = 25    [Parametros.mat]
  Ts = 2    [Parametros.mat]
  uo = 0.5    [Parametros.mat]
(part 1 of 5)
settings Model: SimulationMode=accelerator  Creator=Manu  LastModifiedBy=joaqu
settings SolverCC: AlgebraicLoopSolver=TrustRegion
settings DataIOCC: ReturnWorkspaceOutputs=off
settings OptimizationCC: EfficientMapNaN2IntZero=off
settings DebuggingCC: ArithmeticOperatorsInVariantConditions=warning
settings HardwareCC: TargetBitPerPointer=64.0  TargetBitPerSizeT=64.0  TargetBitPerPtrDiffT=64.0  TargetLongLongMode=on  TargetIntDivRoundTo=Zero  TargetEndianess=LittleEndian  TargetWordSize=64.0  TargetHWDeviceType=MATLAB Host  ProdEqTarget=off
settings SFSimCC: CustomCodeUndefinedFunction=UseInterfaceOnly
settings RTWCC: GPUComputeCapability=3.5
settings CodeAppCC: MaxIdLength=128.0
settings GRTTargetCC: TargetLangStandard=C89/C90 (ANSI)  CombineOutputUpdateFcns=off  GRTInterface=on

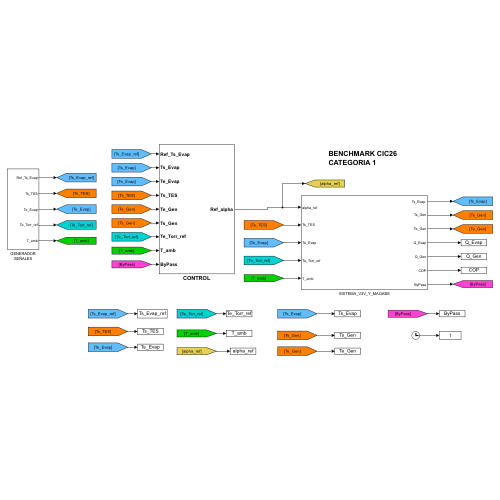
[thumbnail: Simulink's stored preview of the top-level diagram]
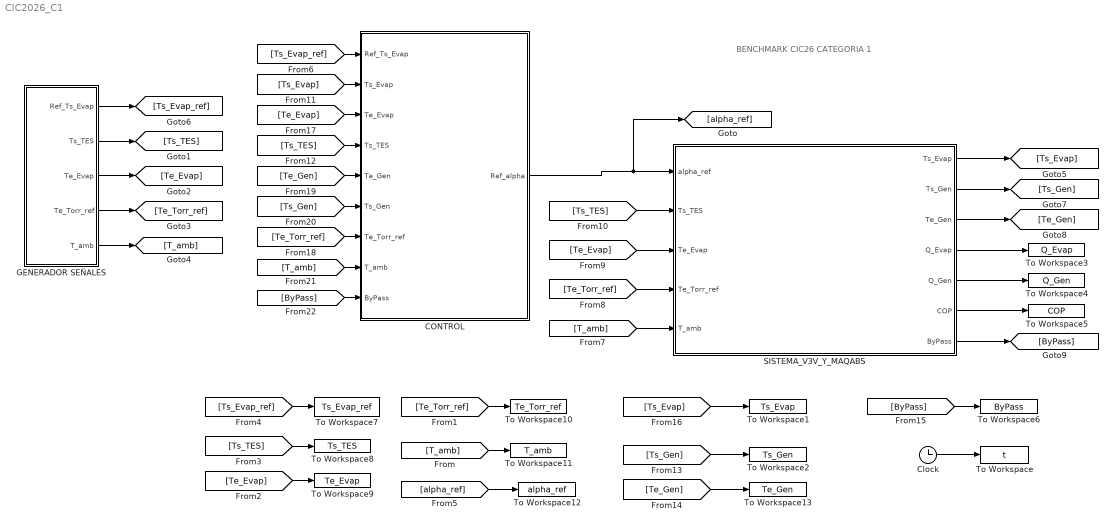
== system CIC2026_C1 ==
  note: BENCHMARK CIC26
      | CATEGORIA 1
  CONTROL : Subsystem
  Clock : Clock
  GENERADOR SEÑALES : Subsystem
  SISTEMA_V3V_Y_MAQABS : Subsystem
  To Workspace : ToWorkspace  VariableName=t  SampleTime=1
  To Workspace1 : ToWorkspace  VariableName=Ts_Evap  SampleTime=1
  To Workspace10 : ToWorkspace  VariableName=Te_Torr_ref  SampleTime=1
  To Workspace11 : ToWorkspace  VariableName=T_amb  SampleTime=1
  To Workspace12 : ToWorkspace  VariableName=alpha_ref  SampleTime=1
  To Workspace13 : ToWorkspace  VariableName=Te_Gen  SampleTime=1
  To Workspace2 : ToWorkspace  VariableName=Ts_Gen  SampleTime=1
  To Workspace3 : ToWorkspace  VariableName=Q_Evap  SampleTime=1
  To Workspace4 : ToWorkspace  VariableName=Q_Gen  SampleTime=1
  To Workspace5 : ToWorkspace  VariableName=COP  SampleTime=1
  To Workspace6 : ToWorkspace  VariableName=ByPass  SampleTime=1
  To Workspace7 : ToWorkspace  VariableName=Ts_Evap_ref  SampleTime=1
  To Workspace8 : ToWorkspace  VariableName=Ts_TES  SampleTime=1
  To Workspace9 : ToWorkspace  VariableName=Te_Evap  SampleTime=1
  wires:
  Clock/1 -> To Workspace/1
  SISTEMA_V3V_Y_MAQABS/1("Ts_Evap ") -> [Ts_Evap]
  SISTEMA_V3V_Y_MAQABS/4(Q_Evap) -> To Workspace3/1
  SISTEMA_V3V_Y_MAQABS/5(Q_Gen) -> To Workspace4/1
  SISTEMA_V3V_Y_MAQABS/6(COP) -> To Workspace5/1
  GENERADOR SEÑALES/1(Ref_Ts_Evap) -> [Ts_Evap_ref]
  GENERADOR SEÑALES/2(Ts_TES) -> [Ts_TES]
  GENERADOR SEÑALES/3(Te_Evap) -> [Te_Evap]
  GENERADOR SEÑALES/4(Te_Torr_ref) -> [Te_Torr_ref]
  GENERADOR SEÑALES/5(T_amb) -> [T_amb]
  [T_amb] -> To Workspace11/1
  [Te_Torr_ref] -> To Workspace10/1
  [Te_Evap] -> To Workspace9/1
  [Ts_TES] -> To Workspace8/1
  [Ts_Evap_ref] -> To Workspace7/1
  [alpha_ref] -> To Workspace12/1
  [T_amb] -> SISTEMA_V3V_Y_MAQABS/5(T_amb)
  [Te_Torr_ref] -> SISTEMA_V3V_Y_MAQABS/4(Te_Torr_ref)
  [Te_Evap] -> SISTEMA_V3V_Y_MAQABS/3(Te_Evap)
  [Ts_TES] -> SISTEMA_V3V_Y_MAQABS/2(Ts_TES)
  [Ts_Evap_ref] -> CONTROL/1(Ref_Ts_Evap)
  [Ts_Evap] -> CONTROL/2(Ts_Evap)
  CONTROL/1(Ref_alpha) -> [alpha_ref], SISTEMA_V3V_Y_MAQABS/1(alpha_ref)
  SISTEMA_V3V_Y_MAQABS/2(Ts_Gen) -> [Ts_Gen]
  [Ts_Gen] -> To Workspace2/1
  SISTEMA_V3V_Y_MAQABS/3(Te_Gen) -> [Te_Gen]
  [Te_Gen] -> To Workspace13/1
  SISTEMA_V3V_Y_MAQABS/7(ByPass) -> [ByPass]
  [ByPass] -> To Workspace6/1
  [Ts_Evap] -> To Workspace1/1
  [Ts_TES] -> CONTROL/4(Ts_TES)
  [Te_Evap] -> CONTROL/3(Te_Evap)
  [Te_Torr_ref] -> CONTROL/7(Te_Torr_ref)
  [Te_Gen] -> CONTROL/5(Te_Gen)
  [Ts_Gen] -> CONTROL/6(Ts_Gen)
  [T_amb] -> CONTROL/8(T_amb)
  [ByPass] -> CONTROL/9(ByPass)
